simulink model "MMC_indc"  (R2026a)
settings: Solver=VariableStepAuto  StopTime=10
model workspace (MAT data in the model file):
  L_arm = 40
  L_arm_pow_rat = 14.4
  L_arm_res = 0.4
  L_arm_satcurrent = 7
  L_tolr = 15
  N = 8
  Rarm = 1
  Vdc = 375.5
libraries: nesl_utility x155, fl_lib x111, ee_lib x107
(part 1 of 14)
settings Model: Creator=tanus  LastModifiedBy=Shefali Pawgi
settings SimscapeCC: SimscapeNominalValues="[{\"value\":\"1\",\"unit\":\"A\"},{\"value\":\"1\",\"unit\":\"bar\"},{\"value\":\"1\",\"unit\":\"cm^2\"},{\"value\":\"1\",\"unit\":\"cm^3/s\"},{\"value\":\"1\",\"unit\":\"kJ/kg\"},{\"value\":\"1\",\"unit\":\"kW\"},{\"value\":\"1\",\"unit\":\"l\"},{\"value\":\"1\",\"unit\":\"N\"},{\"value\":\"1\",\"unit\":\"N*m\"},{\"value\":\"1\",\"unit\":\"V\"}]"  SimscapeLogType=none  SimscapeLogDataHistory=5000.0

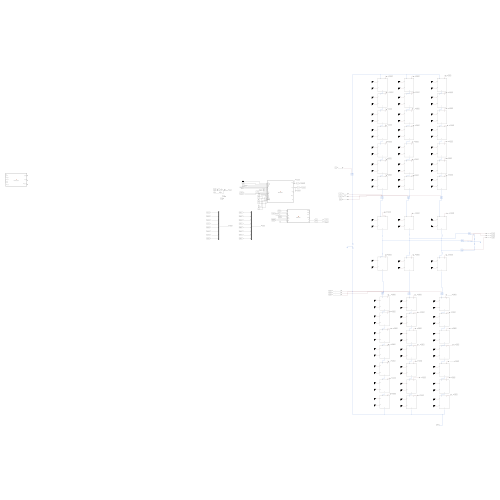
[thumbnail: Simulink's stored preview of the top-level diagram]
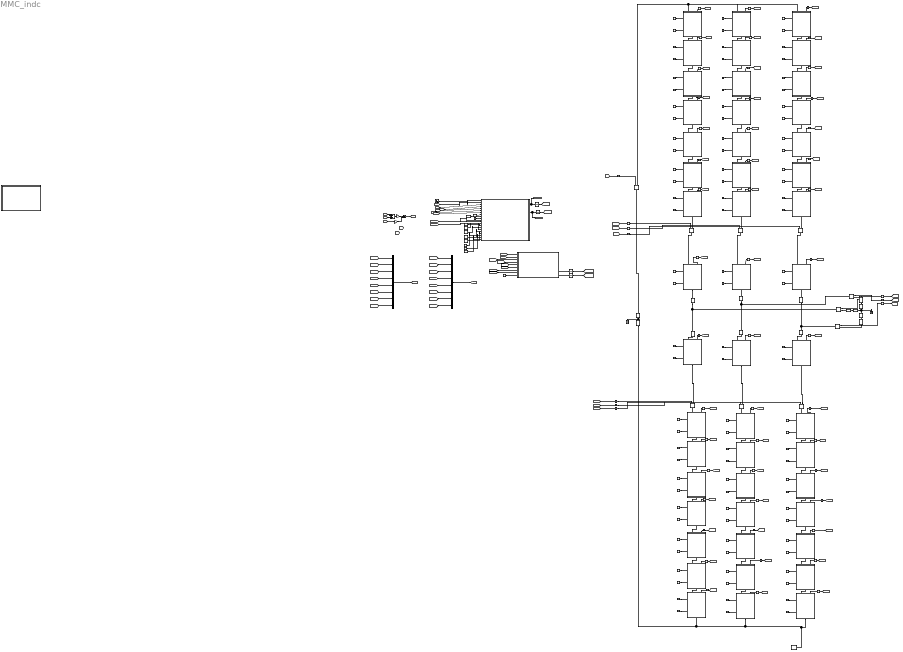
== system MMC_indc ==
  Constant : Constant  Value=Vdc
  Constant1 : Constant  Value=N
  Constant10 : Constant  Value=0.3
  Constant11 : Constant  Value=8
  Constant2 : Constant  Value=20e-3
  Constant3 : Constant  Value=10
  Constant4 : Constant  Value=220e-6
  Constant5 : Constant  Value=0.04
  Constant6 : Constant  Value=100e-3
  Constant7 : Constant
  Constant8 : Constant  Value=0.1
  Constant9 : Constant  Value=0.1
  Current Sensor{,1..9} (10 alike) : fl_lib/Electrical/Electrical Sensors/Current Sensor
  Electrical Reference : fl_lib/Electrical/Electrical Elements/Electrical Reference
  Electrical Reference1 : fl_lib/Electrical/Electrical Elements/Electrical Reference
  Gain : Gain  Gain=0.5
  Gain1 : Gain  Gain=1/3
  Inductor{1..4,6..7} (6 alike) : ee_lib/Passive/Inductor  l=L_arm mH  enable_L_tol=ee.enum.toleranceApplication.applyRand  L_tol=L_tolr  tol_distribution=ee.enum.toleranceDistribution.uniform  nSigma=4  r=L_arm_res Ohm  g=1e-9 1/Ohm  enable_operating_limits=ee.enum.enable.yes  operating_limit_action=ee.enum.passive.reportOpLim.warn  max_working_current=L_arm_satcurrent A  power_rating=L_arm_pow_rat W  i_L_specify=on  i_L_priority=High  i_L=0.44 A  i_L_nominal_specify=off  i_L_nominal_value=1  i_L_nominal_unit=A
  Inductor5 : ee_lib/Passive/Inductor  l=20e-3 H  enable_L_tol=ee.enum.toleranceApplication.none  L_tol=20  tol_distribution=ee.enum.toleranceDistribution.uniform  nSigma=4  r=0 Ohm  g=1e-9 1/Ohm  enable_operating_limits=ee.enum.enable.no  operating_limit_action=ee.enum.passive.reportOpLim.warn  max_working_current=1 A  power_rating=1 W  i_L_specify=on  i_L_priority=High  i_L=0.44 A  i_L_nominal_specify=off  i_L_nominal_value=1  i_L_nominal_unit=A
  Inductor8 : ee_lib/Passive/Inductor  l=20e-3 H  enable_L_tol=ee.enum.toleranceApplication.none  L_tol=20  tol_distribution=ee.enum.toleranceDistribution.uniform  nSigma=4  r=0 Ohm  g=1e-9 1/Ohm  enable_operating_limits=ee.enum.enable.no  operating_limit_action=ee.enum.passive.reportOpLim.warn  max_working_current=1 A  power_rating=1 W  i_L_specify=on  i_L_priority=High  i_L=0.44 A  i_L_nominal_specify=off  i_L_nominal_value=1  i_L_nominal_unit=A
  Inductor9 : ee_lib/Passive/Inductor  l=20e-3 H  enable_L_tol=ee.enum.toleranceApplication.none  L_tol=20  tol_distribution=ee.enum.toleranceDistribution.uniform  nSigma=4  r=0 Ohm  g=1e-9 1/Ohm  enable_operating_limits=ee.enum.enable.no  operating_limit_action=ee.enum.passive.reportOpLim.warn  max_working_current=1 A  power_rating=1 W  i_L_specify=on  i_L_priority=High  i_L=0.44 A  i_L_nominal_specify=off  i_L_nominal_value=1  i_L_nominal_unit=A
  MATLAB Function : MATLAB Function  TreatAsAtomicUnit=on
  MATLAB Function1 : MATLAB Function  TreatAsAtomicUnit=on
  MATLAB Function2 : MATLAB Function  TreatAsAtomicUnit=on
  Mux : Mux  Inputs=8
  Mux1 : Mux  Inputs=8
  PS-Simulink Converter{,1..57} (58 alike) : nesl_utility/PS-Simulink Converter  PhysicalDomain=network_engine_domain  SubClassName=ps_output  LeftPortType=input  RightPortType=output  PseudoPeriodic=off  Frequencies=[]  VectorFormat=inherit  Unit=inherit  AffineConversion=off
  Rarm : Constant  Value=0.4
  Resistor : fl_lib/Electrical/Electrical Elements/Resistor  R=10 Ohm  i_specify=off  i_priority=None  i=0 A  i_nominal_specify=off  i_nominal_value=1  i_nominal_unit=A  v_specify=off  v_priority=None  v=0 V  v_nominal_specify=off  v_nominal_value=1  v_nominal_unit=V
  Resistor1 : fl_lib/Electrical/Electrical Elements/Resistor  R=10 Ohm  i_specify=off  i_priority=None  i=0 A  i_nominal_specify=off  i_nominal_value=1  i_nominal_unit=A  v_specify=off  v_priority=None  v=0 V  v_nominal_specify=off  v_nominal_value=1  v_nominal_unit=V
  Resistor2 : fl_lib/Electrical/Electrical Elements/Resistor  R=10 Ohm  i_specify=off  i_priority=None  i=0 A  i_nominal_specify=off  i_nominal_value=1  i_nominal_unit=A  v_specify=off  v_priority=None  v=0 V  v_nominal_specify=off  v_nominal_value=1  v_nominal_unit=V
  Simulink-PS Converter{3..4,7..8,10..25,27..28,30..38,40..64,66..71,73..77,79..82,84..108} (96 alike) : nesl_utility/Simulink-PS Converter  PhysicalDomain=network_engine_domain  SubClassName=ps_input  LeftPortType=input  RightPortType=output  PseudoPeriodic=off  Frequencies=[]  NoiseDistribution=none  NoiseParameters=[]  Unit=1  AffineConversion=off  FilteringAndDerivatives=provide  SimscapeFilterOrder=1  InputFilterTimeConstant=0.001  UdotUserProvided=0
  Solver Configuration1 : nesl_utility/Solver Configuration  PhysicalDomain=network_engine_domain  SubClassName=solver  LeftPortType=input  RightPortType=generic  Tones=[]  Harmonics=[]  SimulateNoise=off  Profile=off  UseLocalSampling=off  EnableSwitchedLinearOptims=on  FrequencyDomain=off  UseCCode=off  RelTol=0.001  AbsTol=0.001  MinStep=1e-09  ToWorkspace=off  RevertToSquareIcSolve=off  NumHomotopyIterations=100  PhasorMode=off  PhasorModeNumHarmonics=1  ConsistencySolver=NEWTON_XTOL_AFTER_FTOL  CanonicalOrdering=UNORDERED  OptimizeIntermediates=UNOPTIMIZED  IndexReductionMethod=DerivativeReplacement  DoDC=off  ResidualTolerance=1e-09  ConsistencyTolSource=GLOBAL  ConsistencyAbsTol=0.001  ConsistencyRelTol=0.001  ConsistencyTolFactor=0.001  UseLocalSolver=off  LocalSolverChoice=NE_BACKWARD_EULER_ADVANCER  ResolveIndetEquations=on  FunctionEvalNumThread=1  LocalSolverSampleTime=0.001  DoFixedCost=off  MaxNonlinIter=3  MaxModeIter=2  ComputeImpulses=off  ImpulseIterations=2  LinearAlgebra=auto  LinearAlgebraNumThread=0  EquationFormulation=NE_TIME_EF  DelaysMemoryBudget=1024  AutomaticFiltering=on  FilteringTimeConstant=0.001  PartitionStorageMethod=AS_NEEDED  PartitionMemoryBudget=1024  PartitionMethod=ROBUST  MultibodyUseLocalSolver=off  MultibodyLocalSolverChoice=ODE1  MultibodyLocalSolverSampleTime=0.001
  Subsystem1 : Subsystem
      settings: PortSchema="{\"entries\":[{\"content\":{\"sides\":[{\"content\":{\"connectorIds\":[\"LConn1\",\"LConn2\"]},\"type\":\"ConnectorPlacement.EquallySpacedRectSide\",\"uuid\":\"15b6a701-c482-4ab4-b894-e969b74b8fe7\"},{\"content\":{\"side\":\"RIGHT\"},\"type\":\"ConnectorPlacement.EquallySpacedRectSide\",\"uuid\":\"d0e695dd-06b6-4831-9b12-69abc92aa4b4\"},{\"content\":{\"connectorIds\":[\"LConn3\",\"LConn4\"],\"side\":\"TOP\"},\"type\":\"ConnectorPlacement.EquallySpacedRectSide\",\"uuid\":\"2d8cca64-5216-4108-8582-3d735b4d6af0\"},{\"content\":{\"connectorIds\":[\"RConn1\"],\"side\":\"BOTTOM\"},\"type\":\"ConnectorPlacement.EquallySpacedRectSide\",\"uuid\":\"da22ed5b-3a7b-44e1-acef-3ebda742cad5\"}]},\"type\":\"ConnectorPlacement.EquallySpacedConnector\",\"uuid\":\"49f96526-0040-486f-9e93-d2a8b3aa1224\"}],\"packageUris\":[\"http://schema.mathworks.com/mf0/Connector/R2020b\"],\"version\":\"1.0\"}"
  Subsystem10 : Subsystem
      settings: PortSchema="{\"entries\":[{\"content\":{\"sides\":[{\"content\":{\"connectorIds\":[\"LConn1\",\"LConn2\"]},\"type\":\"ConnectorPlacement.EquallySpacedRectSide\",\"uuid\":\"15b6a701-c482-4ab4-b894-e969b74b8fe7\"},{\"content\":{\"side\":\"RIGHT\"},\"type\":\"ConnectorPlacement.EquallySpacedRectSide\",\"uuid\":\"d0e695dd-06b6-4831-9b12-69abc92aa4b4\"},{\"content\":{\"connectorIds\":[\"LConn3\",\"LConn4\"],\"side\":\"TOP\"},\"type\":\"ConnectorPlacement.EquallySpacedRectSide\",\"uuid\":\"2d8cca64-5216-4108-8582-3d735b4d6af0\"},{\"content\":{\"connectorIds\":[\"RConn1\"],\"side\":\"BOTTOM\"},\"type\":\"ConnectorPlacement.EquallySpacedRectSide\",\"uuid\":\"da22ed5b-3a7b-44e1-acef-3ebda742cad5\"}]},\"type\":\"ConnectorPlacement.EquallySpacedConnector\",\"uuid\":\"49f96526-0040-486f-9e93-d2a8b3aa1224\"}],\"packageUris\":[\"http://schema.mathworks.com/mf0/Connector/R2020b\"],\"version\":\"1.0\"}"
  Subsystem11 : Subsystem
      settings: PortSchema="{\"entries\":[{\"content\":{\"sides\":[{\"content\":{\"connectorIds\":[\"LConn1\",\"LConn2\"]},\"type\":\"ConnectorPlacement.EquallySpacedRectSide\",\"uuid\":\"15b6a701-c482-4ab4-b894-e969b74b8fe7\"},{\"content\":{\"side\":\"RIGHT\"},\"type\":\"ConnectorPlacement.EquallySpacedRectSide\",\"uuid\":\"d0e695dd-06b6-4831-9b12-69abc92aa4b4\"},{\"content\":{\"connectorIds\":[\"LConn3\",\"LConn4\"],\"side\":\"TOP\"},\"type\":\"ConnectorPlacement.EquallySpacedRectSide\",\"uuid\":\"2d8cca64-5216-4108-8582-3d735b4d6af0\"},{\"content\":{\"connectorIds\":[\"RConn1\"],\"side\":\"BOTTOM\"},\"type\":\"ConnectorPlacement.EquallySpacedRectSide\",\"uuid\":\"da22ed5b-3a7b-44e1-acef-3ebda742cad5\"}]},\"type\":\"ConnectorPlacement.EquallySpacedConnector\",\"uuid\":\"49f96526-0040-486f-9e93-d2a8b3aa1224\"}],\"packageUris\":[\"http://schema.mathworks.com/mf0/Connector/R2020b\"],\"version\":\"1.0\"}"
  Subsystem12 : Subsystem
      settings: PortSchema="{\"entries\":[{\"content\":{\"sides\":[{\"content\":{\"connectorIds\":[\"LConn1\",\"LConn2\"]},\"type\":\"ConnectorPlacement.EquallySpacedRectSide\",\"uuid\":\"15b6a701-c482-4ab4-b894-e969b74b8fe7\"},{\"content\":{\"side\":\"RIGHT\"},\"type\":\"ConnectorPlacement.EquallySpacedRectSide\",\"uuid\":\"d0e695dd-06b6-4831-9b12-69abc92aa4b4\"},{\"content\":{\"connectorIds\":[\"LConn3\",\"LConn4\"],\"side\":\"TOP\"},\"type\":\"ConnectorPlacement.EquallySpacedRectSide\",\"uuid\":\"2d8cca64-5216-4108-8582-3d735b4d6af0\"},{\"content\":{\"connectorIds\":[\"RConn1\"],\"side\":\"BOTTOM\"},\"type\":\"ConnectorPlacement.EquallySpacedRectSide\",\"uuid\":\"da22ed5b-3a7b-44e1-acef-3ebda742cad5\"}]},\"type\":\"ConnectorPlacement.EquallySpacedConnector\",\"uuid\":\"49f96526-0040-486f-9e93-d2a8b3aa1224\"}],\"packageUris\":[\"http://schema.mathworks.com/mf0/Connector/R2020b\"],\"version\":\"1.0\"}"
  Subsystem13 : Subsystem
      settings: PortSchema="{\"entries\":[{\"content\":{\"sides\":[{\"content\":{\"connectorIds\":[\"LConn1\",\"LConn2\"]},\"type\":\"ConnectorPlacement.EquallySpacedRectSide\",\"uuid\":\"15b6a701-c482-4ab4-b894-e969b74b8fe7\"},{\"content\":{\"side\":\"RIGHT\"},\"type\":\"ConnectorPlacement.EquallySpacedRectSide\",\"uuid\":\"d0e695dd-06b6-4831-9b12-69abc92aa4b4\"},{\"content\":{\"connectorIds\":[\"LConn3\",\"LConn4\"],\"side\":\"TOP\"},\"type\":\"ConnectorPlacement.EquallySpacedRectSide\",\"uuid\":\"2d8cca64-5216-4108-8582-3d735b4d6af0\"},{\"content\":{\"connectorIds\":[\"RConn1\"],\"side\":\"BOTTOM\"},\"type\":\"ConnectorPlacement.EquallySpacedRectSide\",\"uuid\":\"da22ed5b-3a7b-44e1-acef-3ebda742cad5\"}]},\"type\":\"ConnectorPlacement.EquallySpacedConnector\",\"uuid\":\"49f96526-0040-486f-9e93-d2a8b3aa1224\"}],\"packageUris\":[\"http://schema.mathworks.com/mf0/Connector/R2020b\"],\"version\":\"1.0\"}"
  Subsystem14 : Subsystem
      settings: PortSchema="{\"entries\":[{\"content\":{\"sides\":[{\"content\":{\"connectorIds\":[\"LConn1\",\"LConn2\"]},\"type\":\"ConnectorPlacement.EquallySpacedRectSide\",\"uuid\":\"15b6a701-c482-4ab4-b894-e969b74b8fe7\"},{\"content\":{\"side\":\"RIGHT\"},\"type\":\"ConnectorPlacement.EquallySpacedRectSide\",\"uuid\":\"d0e695dd-06b6-4831-9b12-69abc92aa4b4\"},{\"content\":{\"connectorIds\":[\"LConn3\",\"LConn4\"],\"side\":\"TOP\"},\"type\":\"ConnectorPlacement.EquallySpacedRectSide\",\"uuid\":\"2d8cca64-5216-4108-8582-3d735b4d6af0\"},{\"content\":{\"connectorIds\":[\"RConn1\"],\"side\":\"BOTTOM\"},\"type\":\"ConnectorPlacement.EquallySpacedRectSide\",\"uuid\":\"da22ed5b-3a7b-44e1-acef-3ebda742cad5\"}]},\"type\":\"ConnectorPlacement.EquallySpacedConnector\",\"uuid\":\"49f96526-0040-486f-9e93-d2a8b3aa1224\"}],\"packageUris\":[\"http://schema.mathworks.com/mf0/Connector/R2020b\"],\"version\":\"1.0\"}"
  Subsystem16 : Subsystem
      settings: PortSchema="{\"entries\":[{\"content\":{\"sides\":[{\"content\":{\"connectorIds\":[\"LConn1\",\"LConn2\"]},\"type\":\"ConnectorPlacement.EquallySpacedRectSide\",\"uuid\":\"15b6a701-c482-4ab4-b894-e969b74b8fe7\"},{\"content\":{\"side\":\"RIGHT\"},\"type\":\"ConnectorPlacement.EquallySpacedRectSide\",\"uuid\":\"d0e695dd-06b6-4831-9b12-69abc92aa4b4\"},{\"content\":{\"connectorIds\":[\"LConn3\",\"LConn4\"],\"side\":\"TOP\"},\"type\":\"ConnectorPlacement.EquallySpacedRectSide\",\"uuid\":\"2d8cca64-5216-4108-8582-3d735b4d6af0\"},{\"content\":{\"connectorIds\":[\"RConn1\"],\"side\":\"BOTTOM\"},\"type\":\"ConnectorPlacement.EquallySpacedRectSide\",\"uuid\":\"da22ed5b-3a7b-44e1-acef-3ebda742cad5\"}]},\"type\":\"ConnectorPlacement.EquallySpacedConnector\",\"uuid\":\"49f96526-0040-486f-9e93-d2a8b3aa1224\"}],\"packageUris\":[\"http://schema.mathworks.com/mf0/Connector/R2020b\"],\"version\":\"1.0\"}"
  Subsystem17 : Subsystem
      settings: PortSchema="{\"entries\":[{\"content\":{\"sides\":[{\"content\":{\"connectorIds\":[\"LConn1\",\"LConn2\"]},\"type\":\"ConnectorPlacement.EquallySpacedRectSide\",\"uuid\":\"15b6a701-c482-4ab4-b894-e969b74b8fe7\"},{\"content\":{\"side\":\"RIGHT\"},\"type\":\"ConnectorPlacement.EquallySpacedRectSide\",\"uuid\":\"d0e695dd-06b6-4831-9b12-69abc92aa4b4\"},{\"content\":{\"connectorIds\":[\"LConn3\",\"LConn4\"],\"side\":\"TOP\"},\"type\":\"ConnectorPlacement.EquallySpacedRectSide\",\"uuid\":\"2d8cca64-5216-4108-8582-3d735b4d6af0\"},{\"content\":{\"connectorIds\":[\"RConn1\"],\"side\":\"BOTTOM\"},\"type\":\"ConnectorPlacement.EquallySpacedRectSide\",\"uuid\":\"da22ed5b-3a7b-44e1-acef-3ebda742cad5\"}]},\"type\":\"ConnectorPlacement.EquallySpacedConnector\",\"uuid\":\"49f96526-0040-486f-9e93-d2a8b3aa1224\"}],\"packageUris\":[\"http://schema.mathworks.com/mf0/Connector/R2020b\"],\"version\":\"1.0\"}"
  Subsystem18 : Subsystem
      settings: PortSchema="{\"entries\":[{\"content\":{\"sides\":[{\"content\":{\"connectorIds\":[\"LConn1\",\"LConn2\"]},\"type\":\"ConnectorPlacement.EquallySpacedRectSide\",\"uuid\":\"15b6a701-c482-4ab4-b894-e969b74b8fe7\"},{\"content\":{\"side\":\"RIGHT\"},\"type\":\"ConnectorPlacement.EquallySpacedRectSide\",\"uuid\":\"d0e695dd-06b6-4831-9b12-69abc92aa4b4\"},{\"content\":{\"connectorIds\":[\"LConn3\",\"LConn4\"],\"side\":\"TOP\"},\"type\":\"ConnectorPlacement.EquallySpacedRectSide\",\"uuid\":\"2d8cca64-5216-4108-8582-3d735b4d6af0\"},{\"content\":{\"connectorIds\":[\"RConn1\"],\"side\":\"BOTTOM\"},\"type\":\"ConnectorPlacement.EquallySpacedRectSide\",\"uuid\":\"da22ed5b-3a7b-44e1-acef-3ebda742cad5\"}]},\"type\":\"ConnectorPlacement.EquallySpacedConnector\",\"uuid\":\"49f96526-0040-486f-9e93-d2a8b3aa1224\"}],\"packageUris\":[\"http://schema.mathworks.com/mf0/Connector/R2020b\"],\"version\":\"1.0\"}"
  Subsystem19 : Subsystem
      settings: PortSchema="{\"entries\":[{\"content\":{\"sides\":[{\"content\":{\"connectorIds\":[\"LConn1\",\"LConn2\"]},\"type\":\"ConnectorPlacement.EquallySpacedRectSide\",\"uuid\":\"15b6a701-c482-4ab4-b894-e969b74b8fe7\"},{\"content\":{\"side\":\"RIGHT\"},\"type\":\"ConnectorPlacement.EquallySpacedRectSide\",\"uuid\":\"d0e695dd-06b6-4831-9b12-69abc92aa4b4\"},{\"content\":{\"connectorIds\":[\"LConn3\",\"LConn4\"],\"side\":\"TOP\"},\"type\":\"ConnectorPlacement.EquallySpacedRectSide\",\"uuid\":\"2d8cca64-5216-4108-8582-3d735b4d6af0\"},{\"content\":{\"connectorIds\":[\"RConn1\"],\"side\":\"BOTTOM\"},\"type\":\"ConnectorPlacement.EquallySpacedRectSide\",\"uuid\":\"da22ed5b-3a7b-44e1-acef-3ebda742cad5\"}]},\"type\":\"ConnectorPlacement.EquallySpacedConnector\",\"uuid\":\"49f96526-0040-486f-9e93-d2a8b3aa1224\"}],\"packageUris\":[\"http://schema.mathworks.com/mf0/Connector/R2020b\"],\"version\":\"1.0\"}"
  Subsystem2 : Subsystem
      settings: PortSchema="{\"entries\":[{\"content\":{\"sides\":[{\"content\":{\"connectorIds\":[\"LConn1\",\"LConn2\"]},\"type\":\"ConnectorPlacement.EquallySpacedRectSide\",\"uuid\":\"15b6a701-c482-4ab4-b894-e969b74b8fe7\"},{\"content\":{\"side\":\"RIGHT\"},\"type\":\"ConnectorPlacement.EquallySpacedRectSide\",\"uuid\":\"d0e695dd-06b6-4831-9b12-69abc92aa4b4\"},{\"content\":{\"connectorIds\":[\"LConn3\",\"LConn4\"],\"side\":\"TOP\"},\"type\":\"ConnectorPlacement.EquallySpacedRectSide\",\"uuid\":\"2d8cca64-5216-4108-8582-3d735b4d6af0\"},{\"content\":{\"connectorIds\":[\"RConn1\"],\"side\":\"BOTTOM\"},\"type\":\"ConnectorPlacement.EquallySpacedRectSide\",\"uuid\":\"da22ed5b-3a7b-44e1-acef-3ebda742cad5\"}]},\"type\":\"ConnectorPlacement.EquallySpacedConnector\",\"uuid\":\"49f96526-0040-486f-9e93-d2a8b3aa1224\"}],\"packageUris\":[\"http://schema.mathworks.com/mf0/Connector/R2020b\"],\"version\":\"1.0\"}"
  Subsystem20 : Subsystem
      settings: PortSchema="{\"entries\":[{\"content\":{\"sides\":[{\"content\":{\"connectorIds\":[\"LConn1\",\"LConn2\"]},\"type\":\"ConnectorPlacement.EquallySpacedRectSide\",\"uuid\":\"15b6a701-c482-4ab4-b894-e969b74b8fe7\"},{\"content\":{\"side\":\"RIGHT\"},\"type\":\"ConnectorPlacement.EquallySpacedRectSide\",\"uuid\":\"d0e695dd-06b6-4831-9b12-69abc92aa4b4\"},{\"content\":{\"connectorIds\":[\"LConn3\",\"LConn4\"],\"side\":\"TOP\"},\"type\":\"ConnectorPlacement.EquallySpacedRectSide\",\"uuid\":\"2d8cca64-5216-4108-8582-3d735b4d6af0\"},{\"content\":{\"connectorIds\":[\"RConn1\"],\"side\":\"BOTTOM\"},\"type\":\"ConnectorPlacement.EquallySpacedRectSide\",\"uuid\":\"da22ed5b-3a7b-44e1-acef-3ebda742cad5\"}]},\"type\":\"ConnectorPlacement.EquallySpacedConnector\",\"uuid\":\"49f96526-0040-486f-9e93-d2a8b3aa1224\"}],\"packageUris\":[\"http://schema.mathworks.com/mf0/Connector/R2020b\"],\"version\":\"1.0\"}"
  Subsystem21 : Subsystem
      settings: PortSchema="{\"entries\":[{\"content\":{\"sides\":[{\"content\":{\"connectorIds\":[\"LConn1\",\"LConn2\"]},\"type\":\"ConnectorPlacement.EquallySpacedRectSide\",\"uuid\":\"15b6a701-c482-4ab4-b894-e969b74b8fe7\"},{\"content\":{\"side\":\"RIGHT\"},\"type\":\"ConnectorPlacement.EquallySpacedRectSide\",\"uuid\":\"d0e695dd-06b6-4831-9b12-69abc92aa4b4\"},{\"content\":{\"connectorIds\":[\"LConn3\",\"LConn4\"],\"side\":\"TOP\"},\"type\":\"ConnectorPlacement.EquallySpacedRectSide\",\"uuid\":\"2d8cca64-5216-4108-8582-3d735b4d6af0\"},{\"content\":{\"connectorIds\":[\"RConn1\"],\"side\":\"BOTTOM\"},\"type\":\"ConnectorPlacement.EquallySpacedRectSide\",\"uuid\":\"da22ed5b-3a7b-44e1-acef-3ebda742cad5\"}]},\"type\":\"ConnectorPlacement.EquallySpacedConnector\",\"uuid\":\"49f96526-0040-486f-9e93-d2a8b3aa1224\"}],\"packageUris\":[\"http://schema.mathworks.com/mf0/Connector/R2020b\"],\"version\":\"1.0\"}"
  Subsystem22 : Subsystem
      settings: PortSchema="{\"entries\":[{\"content\":{\"sides\":[{\"content\":{\"connectorIds\":[\"LConn1\",\"LConn2\"]},\"type\":\"ConnectorPlacement.EquallySpacedRectSide\",\"uuid\":\"15b6a701-c482-4ab4-b894-e969b74b8fe7\"},{\"content\":{\"side\":\"RIGHT\"},\"type\":\"ConnectorPlacement.EquallySpacedRectSide\",\"uuid\":\"d0e695dd-06b6-4831-9b12-69abc92aa4b4\"},{\"content\":{\"connectorIds\":[\"LConn3\",\"LConn4\"],\"side\":\"TOP\"},\"type\":\"ConnectorPlacement.EquallySpacedRectSide\",\"uuid\":\"2d8cca64-5216-4108-8582-3d735b4d6af0\"},{\"content\":{\"connectorIds\":[\"RConn1\"],\"side\":\"BOTTOM\"},\"type\":\"ConnectorPlacement.EquallySpacedRectSide\",\"uuid\":\"da22ed5b-3a7b-44e1-acef-3ebda742cad5\"}]},\"type\":\"ConnectorPlacement.EquallySpacedConnector\",\"uuid\":\"49f96526-0040-486f-9e93-d2a8b3aa1224\"}],\"packageUris\":[\"http://schema.mathworks.com/mf0/Connector/R2020b\"],\"version\":\"1.0\"}"
  Subsystem23 : Subsystem
      settings: PortSchema="{\"entries\":[{\"content\":{\"sides\":[{\"content\":{\"connectorIds\":[\"LConn1\",\"LConn2\"]},\"type\":\"ConnectorPlacement.EquallySpacedRectSide\",\"uuid\":\"15b6a701-c482-4ab4-b894-e969b74b8fe7\"},{\"content\":{\"side\":\"RIGHT\"},\"type\":\"ConnectorPlacement.EquallySpacedRectSide\",\"uuid\":\"d0e695dd-06b6-4831-9b12-69abc92aa4b4\"},{\"content\":{\"connectorIds\":[\"LConn3\",\"LConn4\"],\"side\":\"TOP\"},\"type\":\"ConnectorPlacement.EquallySpacedRectSide\",\"uuid\":\"2d8cca64-5216-4108-8582-3d735b4d6af0\"},{\"content\":{\"connectorIds\":[\"RConn1\"],\"side\":\"BOTTOM\"},\"type\":\"ConnectorPlacement.EquallySpacedRectSide\",\"uuid\":\"da22ed5b-3a7b-44e1-acef-3ebda742cad5\"}]},\"type\":\"ConnectorPlacement.EquallySpacedConnector\",\"uuid\":\"49f96526-0040-486f-9e93-d2a8b3aa1224\"}],\"packageUris\":[\"http://schema.mathworks.com/mf0/Connector/R2020b\"],\"version\":\"1.0\"}"
  Subsystem24 : Subsystem
      settings: PortSchema="{\"entries\":[{\"content\":{\"sides\":[{\"content\":{\"connectorIds\":[\"LConn1\",\"LConn2\"]},\"type\":\"ConnectorPlacement.EquallySpacedRectSide\",\"uuid\":\"15b6a701-c482-4ab4-b894-e969b74b8fe7\"},{\"content\":{\"side\":\"RIGHT\"},\"type\":\"ConnectorPlacement.EquallySpacedRectSide\",\"uuid\":\"d0e695dd-06b6-4831-9b12-69abc92aa4b4\"},{\"content\":{\"connectorIds\":[\"LConn3\",\"LConn4\"],\"side\":\"TOP\"},\"type\":\"ConnectorPlacement.EquallySpacedRectSide\",\"uuid\":\"2d8cca64-5216-4108-8582-3d735b4d6af0\"},{\"content\":{\"connectorIds\":[\"RConn1\"],\"side\":\"BOTTOM\"},\"type\":\"ConnectorPlacement.EquallySpacedRectSide\",\"uuid\":\"da22ed5b-3a7b-44e1-acef-3ebda742cad5\"}]},\"type\":\"ConnectorPlacement.EquallySpacedConnector\",\"uuid\":\"49f96526-0040-486f-9e93-d2a8b3aa1224\"}],\"packageUris\":[\"http://schema.mathworks.com/mf0/Connector/R2020b\"],\"version\":\"1.0\"}"
  Subsystem25 : Subsystem
      settings: PortSchema="{\"entries\":[{\"content\":{\"sides\":[{\"content\":{\"connectorIds\":[\"LConn1\",\"LConn2\"]},\"type\":\"ConnectorPlacement.EquallySpacedRectSide\",\"uuid\":\"15b6a701-c482-4ab4-b894-e969b74b8fe7\"},{\"content\":{\"side\":\"RIGHT\"},\"type\":\"ConnectorPlacement.EquallySpacedRectSide\",\"uuid\":\"d0e695dd-06b6-4831-9b12-69abc92aa4b4\"},{\"content\":{\"connectorIds\":[\"LConn3\",\"LConn4\"],\"side\":\"TOP\"},\"type\":\"ConnectorPlacement.EquallySpacedRectSide\",\"uuid\":\"2d8cca64-5216-4108-8582-3d735b4d6af0\"},{\"content\":{\"connectorIds\":[\"RConn1\"],\"side\":\"BOTTOM\"},\"type\":\"ConnectorPlacement.EquallySpacedRectSide\",\"uuid\":\"da22ed5b-3a7b-44e1-acef-3ebda742cad5\"}]},\"type\":\"ConnectorPlacement.EquallySpacedConnector\",\"uuid\":\"49f96526-0040-486f-9e93-d2a8b3aa1224\"}],\"packageUris\":[\"http://schema.mathworks.com/mf0/Connector/R2020b\"],\"version\":\"1.0\"}"
  Subsystem26 : Subsystem
      settings: PortSchema="{\"entries\":[{\"content\":{\"sides\":[{\"content\":{\"connectorIds\":[\"LConn1\",\"LConn2\"]},\"type\":\"ConnectorPlacement.EquallySpacedRectSide\",\"uuid\":\"15b6a701-c482-4ab4-b894-e969b74b8fe7\"},{\"content\":{\"side\":\"RIGHT\"},\"type\":\"ConnectorPlacement.EquallySpacedRectSide\",\"uuid\":\"d0e695dd-06b6-4831-9b12-69abc92aa4b4\"},{\"content\":{\"connectorIds\":[\"LConn3\",\"LConn4\"],\"side\":\"TOP\"},\"type\":\"ConnectorPlacement.EquallySpacedRectSide\",\"uuid\":\"2d8cca64-5216-4108-8582-3d735b4d6af0\"},{\"content\":{\"connectorIds\":[\"RConn1\"],\"side\":\"BOTTOM\"},\"type\":\"ConnectorPlacement.EquallySpacedRectSide\",\"uuid\":\"da22ed5b-3a7b-44e1-acef-3ebda742cad5\"}]},\"type\":\"ConnectorPlacement.EquallySpacedConnector\",\"uuid\":\"49f96526-0040-486f-9e93-d2a8b3aa1224\"}],\"packageUris\":[\"http://schema.mathworks.com/mf0/Connector/R2020b\"],\"version\":\"1.0\"}"
  Subsystem27 : Subsystem
      settings: PortSchema="{\"entries\":[{\"content\":{\"sides\":[{\"content\":{\"connectorIds\":[\"LConn1\",\"LConn2\"]},\"type\":\"ConnectorPlacement.EquallySpacedRectSide\",\"uuid\":\"15b6a701-c482-4ab4-b894-e969b74b8fe7\"},{\"content\":{\"side\":\"RIGHT\"},\"type\":\"ConnectorPlacement.EquallySpacedRectSide\",\"uuid\":\"d0e695dd-06b6-4831-9b12-69abc92aa4b4\"},{\"content\":{\"connectorIds\":[\"LConn3\",\"LConn4\"],\"side\":\"TOP\"},\"type\":\"ConnectorPlacement.EquallySpacedRectSide\",\"uuid\":\"2d8cca64-5216-4108-8582-3d735b4d6af0\"},{\"content\":{\"connectorIds\":[\"RConn1\"],\"side\":\"BOTTOM\"},\"type\":\"ConnectorPlacement.EquallySpacedRectSide\",\"uuid\":\"da22ed5b-3a7b-44e1-acef-3ebda742cad5\"}]},\"type\":\"ConnectorPlacement.EquallySpacedConnector\",\"uuid\":\"49f96526-0040-486f-9e93-d2a8b3aa1224\"}],\"packageUris\":[\"http://schema.mathworks.com/mf0/Connector/R2020b\"],\"version\":\"1.0\"}"
  Subsystem28 : Subsystem
      settings: PortSchema="{\"entries\":[{\"content\":{\"sides\":[{\"content\":{\"connectorIds\":[\"LConn1\",\"LConn2\"]},\"type\":\"ConnectorPlacement.EquallySpacedRectSide\",\"uuid\":\"15b6a701-c482-4ab4-b894-e969b74b8fe7\"},{\"content\":{\"side\":\"RIGHT\"},\"type\":\"ConnectorPlacement.EquallySpacedRectSide\",\"uuid\":\"d0e695dd-06b6-4831-9b12-69abc92aa4b4\"},{\"content\":{\"connectorIds\":[\"LConn3\",\"LConn4\"],\"side\":\"TOP\"},\"type\":\"ConnectorPlacement.EquallySpacedRectSide\",\"uuid\":\"2d8cca64-5216-4108-8582-3d735b4d6af0\"},{\"content\":{\"connectorIds\":[\"RConn1\"],\"side\":\"BOTTOM\"},\"type\":\"ConnectorPlacement.EquallySpacedRectSide\",\"uuid\":\"da22ed5b-3a7b-44e1-acef-3ebda742cad5\"}]},\"type\":\"ConnectorPlacement.EquallySpacedConnector\",\"uuid\":\"49f96526-0040-486f-9e93-d2a8b3aa1224\"}],\"packageUris\":[\"http://schema.mathworks.com/mf0/Connector/R2020b\"],\"version\":\"1.0\"}"
  Subsystem3 : Subsystem
      settings: PortSchema="{\"entries\":[{\"content\":{\"sides\":[{\"content\":{\"connectorIds\":[\"LConn1\",\"LConn2\"]},\"type\":\"ConnectorPlacement.EquallySpacedRectSide\",\"uuid\":\"15b6a701-c482-4ab4-b894-e969b74b8fe7\"},{\"content\":{\"side\":\"RIGHT\"},\"type\":\"ConnectorPlacement.EquallySpacedRectSide\",\"uuid\":\"d0e695dd-06b6-4831-9b12-69abc92aa4b4\"},{\"content\":{\"connectorIds\":[\"LConn3\",\"LConn4\"],\"side\":\"TOP\"},\"type\":\"ConnectorPlacement.EquallySpacedRectSide\",\"uuid\":\"2d8cca64-5216-4108-8582-3d735b4d6af0\"},{\"content\":{\"connectorIds\":[\"RConn1\"],\"side\":\"BOTTOM\"},\"type\":\"ConnectorPlacement.EquallySpacedRectSide\",\"uuid\":\"da22ed5b-3a7b-44e1-acef-3ebda742cad5\"}]},\"type\":\"ConnectorPlacement.EquallySpacedConnector\",\"uuid\":\"49f96526-0040-486f-9e93-d2a8b3aa1224\"}],\"packageUris\":[\"http://schema.mathworks.com/mf0/Connector/R2020b\"],\"version\":\"1.0\"}"
  Subsystem30 : Subsystem
      settings: PortSchema="{\"entries\":[{\"content\":{\"sides\":[{\"content\":{\"connectorIds\":[\"LConn1\",\"LConn2\"]},\"type\":\"ConnectorPlacement.EquallySpacedRectSide\",\"uuid\":\"15b6a701-c482-4ab4-b894-e969b74b8fe7\"},{\"content\":{\"side\":\"RIGHT\"},\"type\":\"ConnectorPlacement.EquallySpacedRectSide\",\"uuid\":\"d0e695dd-06b6-4831-9b12-69abc92aa4b4\"},{\"content\":{\"connectorIds\":[\"LConn3\",\"LConn4\"],\"side\":\"TOP\"},\"type\":\"ConnectorPlacement.EquallySpacedRectSide\",\"uuid\":\"2d8cca64-5216-4108-8582-3d735b4d6af0\"},{\"content\":{\"connectorIds\":[\"RConn1\"],\"side\":\"BOTTOM\"},\"type\":\"ConnectorPlacement.EquallySpacedRectSide\",\"uuid\":\"da22ed5b-3a7b-44e1-acef-3ebda742cad5\"}]},\"type\":\"ConnectorPlacement.EquallySpacedConnector\",\"uuid\":\"49f96526-0040-486f-9e93-d2a8b3aa1224\"}],\"packageUris\":[\"http://schema.mathworks.com/mf0/Connector/R2020b\"],\"version\":\"1.0\"}"
  Subsystem31 : Subsystem
      settings: PortSchema="{\"entries\":[{\"content\":{\"sides\":[{\"content\":{\"connectorIds\":[\"LConn1\",\"LConn2\"]},\"type\":\"ConnectorPlacement.EquallySpacedRectSide\",\"uuid\":\"15b6a701-c482-4ab4-b894-e969b74b8fe7\"},{\"content\":{\"side\":\"RIGHT\"},\"type\":\"ConnectorPlacement.EquallySpacedRectSide\",\"uuid\":\"d0e695dd-06b6-4831-9b12-69abc92aa4b4\"},{\"content\":{\"connectorIds\":[\"LConn3\",\"LConn4\"],\"side\":\"TOP\"},\"type\":\"ConnectorPlacement.EquallySpacedRectSide\",\"uuid\":\"2d8cca64-5216-4108-8582-3d735b4d6af0\"},{\"content\":{\"connectorIds\":[\"RConn1\"],\"side\":\"BOTTOM\"},\"type\":\"ConnectorPlacement.EquallySpacedRectSide\",\"uuid\":\"da22ed5b-3a7b-44e1-acef-3ebda742cad5\"}]},\"type\":\"ConnectorPlacement.EquallySpacedConnector\",\"uuid\":\"49f96526-0040-486f-9e93-d2a8b3aa1224\"}],\"packageUris\":[\"http://schema.mathworks.com/mf0/Connector/R2020b\"],\"version\":\"1.0\"}"
  Subsystem33 : Subsystem
      settings: PortSchema="{\"entries\":[{\"content\":{\"sides\":[{\"content\":{\"connectorIds\":[\"LConn1\",\"LConn2\"]},\"type\":\"ConnectorPlacement.EquallySpacedRectSide\",\"uuid\":\"15b6a701-c482-4ab4-b894-e969b74b8fe7\"},{\"content\":{\"side\":\"RIGHT\"},\"type\":\"ConnectorPlacement.EquallySpacedRectSide\",\"uuid\":\"d0e695dd-06b6-4831-9b12-69abc92aa4b4\"},{\"content\":{\"connectorIds\":[\"LConn3\",\"LConn4\"],\"side\":\"TOP\"},\"type\":\"ConnectorPlacement.EquallySpacedRectSide\",\"uuid\":\"2d8cca64-5216-4108-8582-3d735b4d6af0\"},{\"content\":{\"connectorIds\":[\"RConn1\"],\"side\":\"BOTTOM\"},\"type\":\"ConnectorPlacement.EquallySpacedRectSide\",\"uuid\":\"da22ed5b-3a7b-44e1-acef-3ebda742cad5\"}]},\"type\":\"ConnectorPlacement.EquallySpacedConnector\",\"uuid\":\"49f96526-0040-486f-9e93-d2a8b3aa1224\"}],\"packageUris\":[\"http://schema.mathworks.com/mf0/Connector/R2020b\"],\"version\":\"1.0\"}"
  Subsystem34 : Subsystem
      settings: PortSchema="{\"entries\":[{\"content\":{\"sides\":[{\"content\":{\"connectorIds\":[\"LConn1\",\"LConn2\"]},\"type\":\"ConnectorPlacement.EquallySpacedRectSide\",\"uuid\":\"15b6a701-c482-4ab4-b894-e969b74b8fe7\"},{\"content\":{\"side\":\"RIGHT\"},\"type\":\"ConnectorPlacement.EquallySpacedRectSide\",\"uuid\":\"d0e695dd-06b6-4831-9b12-69abc92aa4b4\"},{\"content\":{\"connectorIds\":[\"LConn3\",\"LConn4\"],\"side\":\"TOP\"},\"type\":\"ConnectorPlacement.EquallySpacedRectSide\",\"uuid\":\"2d8cca64-5216-4108-8582-3d735b4d6af0\"},{\"content\":{\"connectorIds\":[\"RConn1\"],\"side\":\"BOTTOM\"},\"type\":\"ConnectorPlacement.EquallySpacedRectSide\",\"uuid\":\"da22ed5b-3a7b-44e1-acef-3ebda742cad5\"}]},\"type\":\"ConnectorPlacement.EquallySpacedConnector\",\"uuid\":\"49f96526-0040-486f-9e93-d2a8b3aa1224\"}],\"packageUris\":[\"http://schema.mathworks.com/mf0/Connector/R2020b\"],\"version\":\"1.0\"}"
  Subsystem35 : Subsystem
      settings: PortSchema="{\"entries\":[{\"content\":{\"sides\":[{\"content\":{\"connectorIds\":[\"LConn1\",\"LConn2\"]},\"type\":\"ConnectorPlacement.EquallySpacedRectSide\",\"uuid\":\"15b6a701-c482-4ab4-b894-e969b74b8fe7\"},{\"content\":{\"side\":\"RIGHT\"},\"type\":\"ConnectorPlacement.EquallySpacedRectSide\",\"uuid\":\"d0e695dd-06b6-4831-9b12-69abc92aa4b4\"},{\"content\":{\"connectorIds\":[\"LConn3\",\"LConn4\"],\"side\":\"TOP\"},\"type\":\"ConnectorPlacement.EquallySpacedRectSide\",\"uuid\":\"2d8cca64-5216-4108-8582-3d735b4d6af0\"},{\"content\":{\"connectorIds\":[\"RConn1\"],\"side\":\"BOTTOM\"},\"type\":\"ConnectorPlacement.EquallySpacedRectSide\",\"uuid\":\"da22ed5b-3a7b-44e1-acef-3ebda742cad5\"}]},\"type\":\"ConnectorPlacement.EquallySpacedConnector\",\"uuid\":\"49f96526-0040-486f-9e93-d2a8b3aa1224\"}],\"packageUris\":[\"http://schema.mathworks.com/mf0/Connector/R2020b\"],\"version\":\"1.0\"}"
  Subsystem36 : Subsystem
      settings: PortSchema="{\"entries\":[{\"content\":{\"sides\":[{\"content\":{\"connectorIds\":[\"LConn1\",\"LConn2\"]},\"type\":\"ConnectorPlacement.EquallySpacedRectSide\",\"uuid\":\"15b6a701-c482-4ab4-b894-e969b74b8fe7\"},{\"content\":{\"side\":\"RIGHT\"},\"type\":\"ConnectorPlacement.EquallySpacedRectSide\",\"uuid\":\"d0e695dd-06b6-4831-9b12-69abc92aa4b4\"},{\"content\":{\"connectorIds\":[\"LConn3\",\"LConn4\"],\"side\":\"TOP\"},\"type\":\"ConnectorPlacement.EquallySpacedRectSide\",\"uuid\":\"2d8cca64-5216-4108-8582-3d735b4d6af0\"},{\"content\":{\"connectorIds\":[\"RConn1\"],\"side\":\"BOTTOM\"},\"type\":\"ConnectorPlacement.EquallySpacedRectSide\",\"uuid\":\"da22ed5b-3a7b-44e1-acef-3ebda742cad5\"}]},\"type\":\"ConnectorPlacement.EquallySpacedConnector\",\"uuid\":\"49f96526-0040-486f-9e93-d2a8b3aa1224\"}],\"packageUris\":[\"http://schema.mathworks.com/mf0/Connector/R2020b\"],\"version\":\"1.0\"}"
  Subsystem37 : Subsystem
      settings: PortSchema="{\"entries\":[{\"content\":{\"sides\":[{\"content\":{\"connectorIds\":[\"LConn1\",\"LConn2\"]},\"type\":\"ConnectorPlacement.EquallySpacedRectSide\",\"uuid\":\"15b6a701-c482-4ab4-b894-e969b74b8fe7\"},{\"content\":{\"side\":\"RIGHT\"},\"type\":\"ConnectorPlacement.EquallySpacedRectSide\",\"uuid\":\"d0e695dd-06b6-4831-9b12-69abc92aa4b4\"},{\"content\":{\"connectorIds\":[\"LConn3\",\"LConn4\"],\"side\":\"TOP\"},\"type\":\"ConnectorPlacement.EquallySpacedRectSide\",\"uuid\":\"2d8cca64-5216-4108-8582-3d735b4d6af0\"},{\"content\":{\"connectorIds\":[\"RConn1\"],\"side\":\"BOTTOM\"},\"type\":\"ConnectorPlacement.EquallySpacedRectSide\",\"uuid\":\"da22ed5b-3a7b-44e1-acef-3ebda742cad5\"}]},\"type\":\"ConnectorPlacement.EquallySpacedConnector\",\"uuid\":\"49f96526-0040-486f-9e93-d2a8b3aa1224\"}],\"packageUris\":[\"http://schema.mathworks.com/mf0/Connector/R2020b\"],\"version\":\"1.0\"}"
  Subsystem38 : Subsystem
      settings: PortSchema="{\"entries\":[{\"content\":{\"sides\":[{\"content\":{\"connectorIds\":[\"LConn1\",\"LConn2\"]},\"type\":\"ConnectorPlacement.EquallySpacedRectSide\",\"uuid\":\"15b6a701-c482-4ab4-b894-e969b74b8fe7\"},{\"content\":{\"side\":\"RIGHT\"},\"type\":\"ConnectorPlacement.EquallySpacedRectSide\",\"uuid\":\"d0e695dd-06b6-4831-9b12-69abc92aa4b4\"},{\"content\":{\"connectorIds\":[\"LConn3\",\"LConn4\"],\"side\":\"TOP\"},\"type\":\"ConnectorPlacement.EquallySpacedRectSide\",\"uuid\":\"2d8cca64-5216-4108-8582-3d735b4d6af0\"},{\"content\":{\"connectorIds\":[\"RConn1\"],\"side\":\"BOTTOM\"},\"type\":\"ConnectorPlacement.EquallySpacedRectSide\",\"uuid\":\"da22ed5b-3a7b-44e1-acef-3ebda742cad5\"}]},\"type\":\"ConnectorPlacement.EquallySpacedConnector\",\"uuid\":\"49f96526-0040-486f-9e93-d2a8b3aa1224\"}],\"packageUris\":[\"http://schema.mathworks.com/mf0/Connector/R2020b\"],\"version\":\"1.0\"}"
  Subsystem39 : Subsystem
      settings: PortSchema="{\"entries\":[{\"content\":{\"sides\":[{\"content\":{\"connectorIds\":[\"LConn1\",\"LConn2\"]},\"type\":\"ConnectorPlacement.EquallySpacedRectSide\",\"uuid\":\"15b6a701-c482-4ab4-b894-e969b74b8fe7\"},{\"content\":{\"side\":\"RIGHT\"},\"type\":\"ConnectorPlacement.EquallySpacedRectSide\",\"uuid\":\"d0e695dd-06b6-4831-9b12-69abc92aa4b4\"},{\"content\":{\"connectorIds\":[\"LConn3\",\"LConn4\"],\"side\":\"TOP\"},\"type\":\"ConnectorPlacement.EquallySpacedRectSide\",\"uuid\":\"2d8cca64-5216-4108-8582-3d735b4d6af0\"},{\"content\":{\"connectorIds\":[\"RConn1\"],\"side\":\"BOTTOM\"},\"type\":\"ConnectorPlacement.EquallySpacedRectSide\",\"uuid\":\"da22ed5b-3a7b-44e1-acef-3ebda742cad5\"}]},\"type\":\"ConnectorPlacement.EquallySpacedConnector\",\"uuid\":\"49f96526-0040-486f-9e93-d2a8b3aa1224\"}],\"packageUris\":[\"http://schema.mathworks.com/mf0/Connector/R2020b\"],\"version\":\"1.0\"}"
  Subsystem40 : Subsystem
      settings: PortSchema="{\"entries\":[{\"content\":{\"sides\":[{\"content\":{\"connectorIds\":[\"LConn1\",\"LConn2\"]},\"type\":\"ConnectorPlacement.EquallySpacedRectSide\",\"uuid\":\"15b6a701-c482-4ab4-b894-e969b74b8fe7\"},{\"content\":{\"side\":\"RIGHT\"},\"type\":\"ConnectorPlacement.EquallySpacedRectSide\",\"uuid\":\"d0e695dd-06b6-4831-9b12-69abc92aa4b4\"},{\"content\":{\"connectorIds\":[\"LConn3\",\"LConn4\"],\"side\":\"TOP\"},\"type\":\"ConnectorPlacement.EquallySpacedRectSide\",\"uuid\":\"2d8cca64-5216-4108-8582-3d735b4d6af0\"},{\"content\":{\"connectorIds\":[\"RConn1\"],\"side\":\"BOTTOM\"},\"type\":\"ConnectorPlacement.EquallySpacedRectSide\",\"uuid\":\"da22ed5b-3a7b-44e1-acef-3ebda742cad5\"}]},\"type\":\"ConnectorPlacement.EquallySpacedConnector\",\"uuid\":\"49f96526-0040-486f-9e93-d2a8b3aa1224\"}],\"packageUris\":[\"http://schema.mathworks.com/mf0/Connector/R2020b\"],\"version\":\"1.0\"}"
  Subsystem41 : Subsystem
      settings: PortSchema="{\"entries\":[{\"content\":{\"sides\":[{\"content\":{\"connectorIds\":[\"LConn1\",\"LConn2\"]},\"type\":\"ConnectorPlacement.EquallySpacedRectSide\",\"uuid\":\"15b6a701-c482-4ab4-b894-e969b74b8fe7\"},{\"content\":{\"side\":\"RIGHT\"},\"type\":\"ConnectorPlacement.EquallySpacedRectSide\",\"uuid\":\"d0e695dd-06b6-4831-9b12-69abc92aa4b4\"},{\"content\":{\"connectorIds\":[\"LConn3\",\"LConn4\"],\"side\":\"TOP\"},\"type\":\"ConnectorPlacement.EquallySpacedRectSide\",\"uuid\":\"2d8cca64-5216-4108-8582-3d735b4d6af0\"},{\"content\":{\"connectorIds\":[\"RConn1\"],\"side\":\"BOTTOM\"},\"type\":\"ConnectorPlacement.EquallySpacedRectSide\",\"uuid\":\"da22ed5b-3a7b-44e1-acef-3ebda742cad5\"}]},\"type\":\"ConnectorPlacement.EquallySpacedConnector\",\"uuid\":\"49f96526-0040-486f-9e93-d2a8b3aa1224\"}],\"packageUris\":[\"http://schema.mathworks.com/mf0/Connector/R2020b\"],\"version\":\"1.0\"}"
  Subsystem42 : Subsystem
      settings: PortSchema="{\"entries\":[{\"content\":{\"sides\":[{\"content\":{\"connectorIds\":[\"LConn1\",\"LConn2\"]},\"type\":\"ConnectorPlacement.EquallySpacedRectSide\",\"uuid\":\"15b6a701-c482-4ab4-b894-e969b74b8fe7\"},{\"content\":{\"side\":\"RIGHT\"},\"type\":\"ConnectorPlacement.EquallySpacedRectSide\",\"uuid\":\"d0e695dd-06b6-4831-9b12-69abc92aa4b4\"},{\"content\":{\"connectorIds\":[\"LConn3\",\"LConn4\"],\"side\":\"TOP\"},\"type\":\"ConnectorPlacement.EquallySpacedRectSide\",\"uuid\":\"2d8cca64-5216-4108-8582-3d735b4d6af0\"},{\"content\":{\"connectorIds\":[\"RConn1\"],\"side\":\"BOTTOM\"},\"type\":\"ConnectorPlacement.EquallySpacedRectSide\",\"uuid\":\"da22ed5b-3a7b-44e1-acef-3ebda742cad5\"}]},\"type\":\"ConnectorPlacement.EquallySpacedConnector\",\"uuid\":\"49f96526-0040-486f-9e93-d2a8b3aa1224\"}],\"packageUris\":[\"http://schema.mathworks.com/mf0/Connector/R2020b\"],\"version\":\"1.0\"}"
  Subsystem43 : Subsystem
      settings: PortSchema="{\"entries\":[{\"content\":{\"sides\":[{\"content\":{\"connectorIds\":[\"LConn1\",\"LConn2\"]},\"type\":\"ConnectorPlacement.EquallySpacedRectSide\",\"uuid\":\"15b6a701-c482-4ab4-b894-e969b74b8fe7\"},{\"content\":{\"side\":\"RIGHT\"},\"type\":\"ConnectorPlacement.EquallySpacedRectSide\",\"uuid\":\"d0e695dd-06b6-4831-9b12-69abc92aa4b4\"},{\"content\":{\"connectorIds\":[\"LConn3\",\"LConn4\"],\"side\":\"TOP\"},\"type\":\"ConnectorPlacement.EquallySpacedRectSide\",\"uuid\":\"2d8cca64-5216-4108-8582-3d735b4d6af0\"},{\"content\":{\"connectorIds\":[\"RConn1\"],\"side\":\"BOTTOM\"},\"type\":\"ConnectorPlacement.EquallySpacedRectSide\",\"uuid\":\"da22ed5b-3a7b-44e1-acef-3ebda742cad5\"}]},\"type\":\"ConnectorPlacement.EquallySpacedConnector\",\"uuid\":\"49f96526-0040-486f-9e93-d2a8b3aa1224\"}],\"packageUris\":[\"http://schema.mathworks.com/mf0/Connector/R2020b\"],\"version\":\"1.0\"}"
  Subsystem44 : Subsystem
      settings: PortSchema="{\"entries\":[{\"content\":{\"sides\":[{\"content\":{\"connectorIds\":[\"LConn1\",\"LConn2\"]},\"type\":\"ConnectorPlacement.EquallySpacedRectSide\",\"uuid\":\"15b6a701-c482-4ab4-b894-e969b74b8fe7\"},{\"content\":{\"side\":\"RIGHT\"},\"type\":\"ConnectorPlacement.EquallySpacedRectSide\",\"uuid\":\"d0e695dd-06b6-4831-9b12-69abc92aa4b4\"},{\"content\":{\"connectorIds\":[\"LConn3\",\"LConn4\"],\"side\":\"TOP\"},\"type\":\"ConnectorPlacement.EquallySpacedRectSide\",\"uuid\":\"2d8cca64-5216-4108-8582-3d735b4d6af0\"},{\"content\":{\"connectorIds\":[\"RConn1\"],\"side\":\"BOTTOM\"},\"type\":\"ConnectorPlacement.EquallySpacedRectSide\",\"uuid\":\"da22ed5b-3a7b-44e1-acef-3ebda742cad5\"}]},\"type\":\"ConnectorPlacement.EquallySpacedConnector\",\"uuid\":\"49f96526-0040-486f-9e93-d2a8b3aa1224\"}],\"packageUris\":[\"http://schema.mathworks.com/mf0/Connector/R2020b\"],\"version\":\"1.0\"}"
  Subsystem45 : Subsystem
      settings: PortSchema="{\"entries\":[{\"content\":{\"sides\":[{\"content\":{\"connectorIds\":[\"LConn1\",\"LConn2\"]},\"type\":\"ConnectorPlacement.EquallySpacedRectSide\",\"uuid\":\"15b6a701-c482-4ab4-b894-e969b74b8fe7\"},{\"content\":{\"side\":\"RIGHT\"},\"type\":\"ConnectorPlacement.EquallySpacedRectSide\",\"uuid\":\"d0e695dd-06b6-4831-9b12-69abc92aa4b4\"},{\"content\":{\"connectorIds\":[\"LConn3\",\"LConn4\"],\"side\":\"TOP\"},\"type\":\"ConnectorPlacement.EquallySpacedRectSide\",\"uuid\":\"2d8cca64-5216-4108-8582-3d735b4d6af0\"},{\"content\":{\"connectorIds\":[\"RConn1\"],\"side\":\"BOTTOM\"},\"type\":\"ConnectorPlacement.EquallySpacedRectSide\",\"uuid\":\"da22ed5b-3a7b-44e1-acef-3ebda742cad5\"}]},\"type\":\"ConnectorPlacement.EquallySpacedConnector\",\"uuid\":\"49f96526-0040-486f-9e93-d2a8b3aa1224\"}],\"packageUris\":[\"http://schema.mathworks.com/mf0/Connector/R2020b\"],\"version\":\"1.0\"}"
  Subsystem46 : Subsystem
      settings: PortSchema="{\"entries\":[{\"content\":{\"sides\":[{\"content\":{\"connectorIds\":[\"LConn1\",\"LConn2\"]},\"type\":\"ConnectorPlacement.EquallySpacedRectSide\",\"uuid\":\"15b6a701-c482-4ab4-b894-e969b74b8fe7\"},{\"content\":{\"side\":\"RIGHT\"},\"type\":\"ConnectorPlacement.EquallySpacedRectSide\",\"uuid\":\"d0e695dd-06b6-4831-9b12-69abc92aa4b4\"},{\"content\":{\"connectorIds\":[\"LConn3\",\"LConn4\"],\"side\":\"TOP\"},\"type\":\"ConnectorPlacement.EquallySpacedRectSide\",\"uuid\":\"2d8cca64-5216-4108-8582-3d735b4d6af0\"},{\"content\":{\"connectorIds\":[\"RConn1\"],\"side\":\"BOTTOM\"},\"type\":\"ConnectorPlacement.EquallySpacedRectSide\",\"uuid\":\"da22ed5b-3a7b-44e1-acef-3ebda742cad5\"}]},\"type\":\"ConnectorPlacement.EquallySpacedConnector\",\"uuid\":\"49f96526-0040-486f-9e93-d2a8b3aa1224\"}],\"packageUris\":[\"http://schema.mathworks.com/mf0/Connector/R2020b\"],\"version\":\"1.0\"}"
  Subsystem47 : Subsystem
      settings: PortSchema="{\"entries\":[{\"content\":{\"sides\":[{\"content\":{\"connectorIds\":[\"LConn1\",\"LConn2\"]},\"type\":\"ConnectorPlacement.EquallySpacedRectSide\",\"uuid\":\"15b6a701-c482-4ab4-b894-e969b74b8fe7\"},{\"content\":{\"side\":\"RIGHT\"},\"type\":\"ConnectorPlacement.EquallySpacedRectSide\",\"uuid\":\"d0e695dd-06b6-4831-9b12-69abc92aa4b4\"},{\"content\":{\"connectorIds\":[\"LConn3\",\"LConn4\"],\"side\":\"TOP\"},\"type\":\"ConnectorPlacement.EquallySpacedRectSide\",\"uuid\":\"2d8cca64-5216-4108-8582-3d735b4d6af0\"},{\"content\":{\"connectorIds\":[\"RConn1\"],\"side\":\"BOTTOM\"},\"type\":\"ConnectorPlacement.EquallySpacedRectSide\",\"uuid\":\"da22ed5b-3a7b-44e1-acef-3ebda742cad5\"}]},\"type\":\"ConnectorPlacement.EquallySpacedConnector\",\"uuid\":\"49f96526-0040-486f-9e93-d2a8b3aa1224\"}],\"packageUris\":[\"http://schema.mathworks.com/mf0/Connector/R2020b\"],\"version\":\"1.0\"}"
  Subsystem48 : Subsystem
      settings: PortSchema="{\"entries\":[{\"content\":{\"sides\":[{\"content\":{\"connectorIds\":[\"LConn1\",\"LConn2\"]},\"type\":\"ConnectorPlacement.EquallySpacedRectSide\",\"uuid\":\"15b6a701-c482-4ab4-b894-e969b74b8fe7\"},{\"content\":{\"side\":\"RIGHT\"},\"type\":\"ConnectorPlacement.EquallySpacedRectSide\",\"uuid\":\"d0e695dd-06b6-4831-9b12-69abc92aa4b4\"},{\"content\":{\"connectorIds\":[\"LConn3\",\"LConn4\"],\"side\":\"TOP\"},\"type\":\"ConnectorPlacement.EquallySpacedRectSide\",\"uuid\":\"2d8cca64-5216-4108-8582-3d735b4d6af0\"},{\"content\":{\"connectorIds\":[\"RConn1\"],\"side\":\"BOTTOM\"},\"type\":\"ConnectorPlacement.EquallySpacedRectSide\",\"uuid\":\"da22ed5b-3a7b-44e1-acef-3ebda742cad5\"}]},\"type\":\"ConnectorPlacement.EquallySpacedConnector\",\"uuid\":\"49f96526-0040-486f-9e93-d2a8b3aa1224\"}],\"packageUris\":[\"http://schema.mathworks.com/mf0/Connector/R2020b\"],\"version\":\"1.0\"}"
  Subsystem49 : Subsystem
      settings: PortSchema="{\"entries\":[{\"content\":{\"sides\":[{\"content\":{\"connectorIds\":[\"LConn1\",\"LConn2\"]},\"type\":\"ConnectorPlacement.EquallySpacedRectSide\",\"uuid\":\"15b6a701-c482-4ab4-b894-e969b74b8fe7\"},{\"content\":{\"side\":\"RIGHT\"},\"type\":\"ConnectorPlacement.EquallySpacedRectSide\",\"uuid\":\"d0e695dd-06b6-4831-9b12-69abc92aa4b4\"},{\"content\":{\"connectorIds\":[\"LConn3\",\"LConn4\"],\"side\":\"TOP\"},\"type\":\"ConnectorPlacement.EquallySpacedRectSide\",\"uuid\":\"2d8cca64-5216-4108-8582-3d735b4d6af0\"},{\"content\":{\"connectorIds\":[\"RConn1\"],\"side\":\"BOTTOM\"},\"type\":\"ConnectorPlacement.EquallySpacedRectSide\",\"uuid\":\"da22ed5b-3a7b-44e1-acef-3ebda742cad5\"}]},\"type\":\"ConnectorPlacement.EquallySpacedConnector\",\"uuid\":\"49f96526-0040-486f-9e93-d2a8b3aa1224\"}],\"packageUris\":[\"http://schema.mathworks.com/mf0/Connector/R2020b\"],\"version\":\"1.0\"}"
  Subsystem51 : Subsystem
      settings: PortSchema="{\"entries\":[{\"content\":{\"sides\":[{\"content\":{\"connectorIds\":[\"LConn1\",\"LConn2\"]},\"type\":\"ConnectorPlacement.EquallySpacedRectSide\",\"uuid\":\"15b6a701-c482-4ab4-b894-e969b74b8fe7\"},{\"content\":{\"side\":\"RIGHT\"},\"type\":\"ConnectorPlacement.EquallySpacedRectSide\",\"uuid\":\"d0e695dd-06b6-4831-9b12-69abc92aa4b4\"},{\"content\":{\"connectorIds\":[\"LConn3\",\"LConn4\"],\"side\":\"TOP\"},\"type\":\"ConnectorPlacement.EquallySpacedRectSide\",\"uuid\":\"2d8cca64-5216-4108-8582-3d735b4d6af0\"},{\"content\":{\"connectorIds\":[\"RConn1\"],\"side\":\"BOTTOM\"},\"type\":\"ConnectorPlacement.EquallySpacedRectSide\",\"uuid\":\"da22ed5b-3a7b-44e1-acef-3ebda742cad5\"}]},\"type\":\"ConnectorPlacement.EquallySpacedConnector\",\"uuid\":\"49f96526-0040-486f-9e93-d2a8b3aa1224\"}],\"packageUris\":[\"http://schema.mathworks.com/mf0/Connector/R2020b\"],\"version\":\"1.0\"}"
  Subsystem52 : Subsystem
      settings: PortSchema="{\"entries\":[{\"content\":{\"sides\":[{\"content\":{\"connectorIds\":[\"LConn1\",\"LConn2\"]},\"type\":\"ConnectorPlacement.EquallySpacedRectSide\",\"uuid\":\"15b6a701-c482-4ab4-b894-e969b74b8fe7\"},{\"content\":{\"side\":\"RIGHT\"},\"type\":\"ConnectorPlacement.EquallySpacedRectSide\",\"uuid\":\"d0e695dd-06b6-4831-9b12-69abc92aa4b4\"},{\"content\":{\"connectorIds\":[\"LConn3\",\"LConn4\"],\"side\":\"TOP\"},\"type\":\"ConnectorPlacement.EquallySpacedRectSide\",\"uuid\":\"2d8cca64-5216-4108-8582-3d735b4d6af0\"},{\"content\":{\"connectorIds\":[\"RConn1\"],\"side\":\"BOTTOM\"},\"type\":\"ConnectorPlacement.EquallySpacedRectSide\",\"uuid\":\"da22ed5b-3a7b-44e1-acef-3ebda742cad5\"}]},\"type\":\"ConnectorPlacement.EquallySpacedConnector\",\"uuid\":\"49f96526-0040-486f-9e93-d2a8b3aa1224\"}],\"packageUris\":[\"http://schema.mathworks.com/mf0/Connector/R2020b\"],\"version\":\"1.0\"}"
  Subsystem53 : Subsystem
      settings: PortSchema="{\"entries\":[{\"content\":{\"sides\":[{\"content\":{\"connectorIds\":[\"LConn1\",\"LConn2\"]},\"type\":\"ConnectorPlacement.EquallySpacedRectSide\",\"uuid\":\"15b6a701-c482-4ab4-b894-e969b74b8fe7\"},{\"content\":{\"side\":\"RIGHT\"},\"type\":\"ConnectorPlacement.EquallySpacedRectSide\",\"uuid\":\"d0e695dd-06b6-4831-9b12-69abc92aa4b4\"},{\"content\":{\"connectorIds\":[\"LConn3\",\"LConn4\"],\"side\":\"TOP\"},\"type\":\"ConnectorPlacement.EquallySpacedRectSide\",\"uuid\":\"2d8cca64-5216-4108-8582-3d735b4d6af0\"},{\"content\":{\"connectorIds\":[\"RConn1\"],\"side\":\"BOTTOM\"},\"type\":\"ConnectorPlacement.EquallySpacedRectSide\",\"uuid\":\"da22ed5b-3a7b-44e1-acef-3ebda742cad5\"}]},\"type\":\"ConnectorPlacement.EquallySpacedConnector\",\"uuid\":\"49f96526-0040-486f-9e93-d2a8b3aa1224\"}],\"packageUris\":[\"http://schema.mathworks.com/mf0/Connector/R2020b\"],\"version\":\"1.0\"}"
  Subsystem54 : Subsystem
      settings: PortSchema="{\"entries\":[{\"content\":{\"sides\":[{\"content\":{\"connectorIds\":[\"LConn1\",\"LConn2\"]},\"type\":\"ConnectorPlacement.EquallySpacedRectSide\",\"uuid\":\"15b6a701-c482-4ab4-b894-e969b74b8fe7\"},{\"content\":{\"side\":\"RIGHT\"},\"type\":\"ConnectorPlacement.EquallySpacedRectSide\",\"uuid\":\"d0e695dd-06b6-4831-9b12-69abc92aa4b4\"},{\"content\":{\"connectorIds\":[\"LConn3\",\"LConn4\"],\"side\":\"TOP\"},\"type\":\"ConnectorPlacement.EquallySpacedRectSide\",\"uuid\":\"2d8cca64-5216-4108-8582-3d735b4d6af0\"},{\"content\":{\"connectorIds\":[\"RConn1\"],\"side\":\"BOTTOM\"},\"type\":\"ConnectorPlacement.EquallySpacedRectSide\",\"uuid\":\"da22ed5b-3a7b-44e1-acef-3ebda742cad5\"}]},\"type\":\"ConnectorPlacement.EquallySpacedConnector\",\"uuid\":\"49f96526-0040-486f-9e93-d2a8b3aa1224\"}],\"packageUris\":[\"http://schema.mathworks.com/mf0/Connector/R2020b\"],\"version\":\"1.0\"}"
  Subsystem6 : Subsystem
      settings: PortSchema="{\"entries\":[{\"content\":{\"sides\":[{\"content\":{\"connectorIds\":[\"LConn1\",\"LConn2\"]},\"type\":\"ConnectorPlacement.EquallySpacedRectSide\",\"uuid\":\"15b6a701-c482-4ab4-b894-e969b74b8fe7\"},{\"content\":{\"side\":\"RIGHT\"},\"type\":\"ConnectorPlacement.EquallySpacedRectSide\",\"uuid\":\"d0e695dd-06b6-4831-9b12-69abc92aa4b4\"},{\"content\":{\"connectorIds\":[\"LConn3\",\"LConn4\"],\"side\":\"TOP\"},\"type\":\"ConnectorPlacement.EquallySpacedRectSide\",\"uuid\":\"2d8cca64-5216-4108-8582-3d735b4d6af0\"},{\"content\":{\"connectorIds\":[\"RConn1\"],\"side\":\"BOTTOM\"},\"type\":\"ConnectorPlacement.EquallySpacedRectSide\",\"uuid\":\"da22ed5b-3a7b-44e1-acef-3ebda742cad5\"}]},\"type\":\"ConnectorPlacement.EquallySpacedConnector\",\"uuid\":\"49f96526-0040-486f-9e93-d2a8b3aa1224\"}],\"packageUris\":[\"http://schema.mathworks.com/mf0/Connector/R2020b\"],\"version\":\"1.0\"}"
  Subsystem7 : Subsystem
      settings: PortSchema="{\"entries\":[{\"content\":{\"sides\":[{\"content\":{\"connectorIds\":[\"LConn1\",\"LConn2\"]},\"type\":\"ConnectorPlacement.EquallySpacedRectSide\",\"uuid\":\"15b6a701-c482-4ab4-b894-e969b74b8fe7\"},{\"content\":{\"side\":\"RIGHT\"},\"type\":\"ConnectorPlacement.EquallySpacedRectSide\",\"uuid\":\"d0e695dd-06b6-4831-9b12-69abc92aa4b4\"},{\"content\":{\"connectorIds\":[\"LConn3\",\"LConn4\"],\"side\":\"TOP\"},\"type\":\"ConnectorPlacement.EquallySpacedRectSide\",\"uuid\":\"2d8cca64-5216-4108-8582-3d735b4d6af0\"},{\"content\":{\"connectorIds\":[\"RConn1\"],\"side\":\"BOTTOM\"},\"type\":\"ConnectorPlacement.EquallySpacedRectSide\",\"uuid\":\"da22ed5b-3a7b-44e1-acef-3ebda742cad5\"}]},\"type\":\"ConnectorPlacement.EquallySpacedConnector\",\"uuid\":\"49f96526-0040-486f-9e93-d2a8b3aa1224\"}],\"packageUris\":[\"http://schema.mathworks.com/mf0/Connector/R2020b\"],\"version\":\"1.0\"}"
  Subsystem8 : Subsystem
      settings: PortSchema="{\"entries\":[{\"content\":{\"sides\":[{\"content\":{\"connectorIds\":[\"LConn1\",\"LConn2\"]},\"type\":\"ConnectorPlacement.EquallySpacedRectSide\",\"uuid\":\"15b6a701-c482-4ab4-b894-e969b74b8fe7\"},{\"content\":{\"side\":\"RIGHT\"},\"type\":\"ConnectorPlacement.EquallySpacedRectSide\",\"uuid\":\"d0e695dd-06b6-4831-9b12-69abc92aa4b4\"},{\"content\":{\"connectorIds\":[\"LConn3\",\"LConn4\"],\"side\":\"TOP\"},\"type\":\"ConnectorPlacement.EquallySpacedRectSide\",\"uuid\":\"2d8cca64-5216-4108-8582-3d735b4d6af0\"},{\"content\":{\"connectorIds\":[\"RConn1\"],\"side\":\"BOTTOM\"},\"type\":\"ConnectorPlacement.EquallySpacedRectSide\",\"uuid\":\"da22ed5b-3a7b-44e1-acef-3ebda742cad5\"}]},\"type\":\"ConnectorPlacement.EquallySpacedConnector\",\"uuid\":\"49f96526-0040-486f-9e93-d2a8b3aa1224\"}],\"packageUris\":[\"http://schema.mathworks.com/mf0/Connector/R2020b\"],\"version\":\"1.0\"}"
  Subsystem9 : Subsystem
      settings: PortSchema="{\"entries\":[{\"content\":{\"sides\":[{\"content\":{\"connectorIds\":[\"LConn1\",\"LConn2\"]},\"type\":\"ConnectorPlacement.EquallySpacedRectSide\",\"uuid\":\"15b6a701-c482-4ab4-b894-e969b74b8fe7\"},{\"content\":{\"side\":\"RIGHT\"},\"type\":\"ConnectorPlacement.EquallySpacedRectSide\",\"uuid\":\"d0e695dd-06b6-4831-9b12-69abc92aa4b4\"},{\"content\":{\"connectorIds\":[\"LConn3\",\"LConn4\"],\"side\":\"TOP\"},\"type\":\"ConnectorPlacement.EquallySpacedRectSide\",\"uuid\":\"2d8cca64-5216-4108-8582-3d735b4d6af0\"},{\"content\":{\"connectorIds\":[\"RConn1\"],\"side\":\"BOTTOM\"},\"type\":\"ConnectorPlacement.EquallySpacedRectSide\",\"uuid\":\"da22ed5b-3a7b-44e1-acef-3ebda742cad5\"}]},\"type\":\"ConnectorPlacement.EquallySpacedConnector\",\"uuid\":\"49f96526-0040-486f-9e93-d2a8b3aa1224\"}],\"packageUris\":[\"http://schema.mathworks.com/mf0/Connector/R2020b\"],\"version\":\"1.0\"}"
  Sum : Sum  Inputs=|++
  Sum1 : Sum  Inputs=+-
  Unit Delay{,1..3} (4 alike) : UnitDelay  SampleTime=-1
  Voltage Source : ee_lib/Sources/Voltage Source  dc_voltage=375.5 V  ac_voltage=0 V  ac_shift=0 rad  ac_frequency=60 Hz  noise_mode=ee.enum.sources.noise.Disabled  PSD=0 V^2/Hz  sample_time=1e-3 s  repeatability=ee.enum.sources.repeatability.NotRepeatable  user_seed=0  auto_seed=3499211588  i_specify=off  i_priority=None  i=0 A  i_nominal_specify=off  i_nominal_value=1  i_nominal_unit=A  v_specify=off  v_priority=None  v=0 V  v_nominal_specify=off  v_nominal_value=1  v_nominal_unit=V
  Voltage Source1 : ee_lib/Sources/Voltage Source  dc_voltage=375.5 V  ac_voltage=0 V  ac_shift=0 rad  ac_frequency=60 Hz  noise_mode=ee.enum.sources.noise.Disabled  PSD=0 V^2/Hz  sample_time=1e-3 s  repeatability=ee.enum.sources.repeatability.NotRepeatable  user_seed=0  auto_seed=2915145293  i_specify=off  i_priority=None  i=0 A  i_nominal_specify=off  i_nominal_value=1  i_nominal_unit=A  v_specify=off  v_priority=None  v=0 V  v_nominal_specify=off  v_nominal_value=1  v_nominal_unit=V
  ia_ref : Sin  Frequency=2*pi*50  SampleTime=0
  tag scope: ia_circ=global, ia_lower=global, ia_meas=global, ia_upper=global, ib_lower=global, ib_meas=global, ib_upper=global, ic_lower=global, ic_meas=global, ic_upper=global, la_SM1_Vc=global, la_SM2_Vc=global, la_SM3_Vc=global, la_SM4_Vc=global, la_SM5_Vc=global, la_SM6_Vc=global, la_SM7_Vc=global, la_SM8_Vc=global, lb_SM1_Vc=global, lb_SM2_Vc=global, lb_SM3_Vc=global, lb_SM4_Vc=global, lb_SM5_Vc=global, lb_SM6_Vc=global, lb_SM7_Vc=global, lb_SM8_Vc=global, lc_SM1_Vc=global, lc_SM2_Vc=global, lc_SM3_Vc=global, lc_SM4_Vc=global, lc_SM5_Vc=global, lc_SM6_Vc=global, lc_SM7_Vc=global, lc_SM8_Vc=global, ua_SM1_Vc=global, ua_SM2_Vc=global, ua_SM3_Vc=global, ua_SM4_Vc=global, ua_SM5_Vc=global, ua_SM6_Vc=global, ua_SM7_Vc=global, ua_SM8_Vc=global, ub_SM1_Vc=global, ub_SM2_Vc=global, ub_SM3_Vc=global, ub_SM4_Vc=global, ub_SM5_Vc=global, ub_SM6_Vc=global, ub_SM7_Vc=global, ub_SM8_Vc=global, uc_SM1_Vc=global, uc_SM2_Vc=global, uc_SM3_Vc=global, uc_SM4_Vc=global, uc_SM5_Vc=global, uc_SM6_Vc=global, uc_SM7_Vc=global, uc_SM8_Vc=global
  wires:
  PS-Simulink Converter10/1 -> [I_dc]  "I_dc"
  PS-Simulink Converter4/1 -> [ia_lower]  "ia_lower"
  PS-Simulink Converter5/1 -> [ib_lower]  "ib_lower"
  PS-Simulink Converter6/1 -> [ic_lower]  "ic_lower"
  PS-Simulink Converter1/1 -> [ia_upper]  "ia_upper"
  PS-Simulink Converter2/1 -> [ib_upper]  "ib_upper"
  PS-Simulink Converter3/1 -> [ic_upper]  "ic_upper"
  PS-Simulink Converter8/1 -> [ia_meas]  "i_a"
  PS-Simulink Converter7/1 -> [ib_meas]  "i_b"
  PS-Simulink Converter9/1 -> [ic_meas]  "i_c"
  Constant/1 -> MATLAB Function1/8(Vdc)
  ia_ref/1 -> MATLAB Function1/1(i_ref)
  Rarm/1 -> MATLAB Function1/15(Rarm)
  Constant1/1 -> MATLAB Function1/10(N)
  Constant2/1 -> MATLAB Function1/16(L_load)
  Constant3/1 -> MATLAB Function1/17(R_load)
  [ia_meas] -> MATLAB Function1/2(i_out_meas)
  [ia_upper] -> MATLAB Function1/4(i_upper)
  [ia_lower] -> MATLAB Function1/5(i_lower)
  [ia_upper] -> Sum/1
  [ia_lower] -> Sum/2
  Sum/1 -> Gain/1
  Gain/1 -> Sum1/1
  [I_dc] -> Gain1/1
  Gain1/1 -> Sum1/2
  Sum1/1 -> [ia_circ]  "ia_circ"
  [ia_circ] -> MATLAB Function1/3(i_circ_meas)
  PS-Simulink Converter/1 -> [ua_SM1_Vc]
  PS-Simulink Converter11/1 -> [ua_SM2_Vc]
  PS-Simulink Converter12/1 -> [ua_SM3_Vc]
  PS-Simulink Converter13/1 -> [ua_SM4_Vc]
  PS-Simulink Converter14/1 -> [ua_SM5_Vc]
  PS-Simulink Converter15/1 -> [ua_SM6_Vc]
  PS-Simulink Converter16/1 -> [ua_SM7_Vc]
  PS-Simulink Converter17/1 -> [ua_SM8_Vc]
  PS-Simulink Converter18/1 -> [ub_SM8_Vc]
  PS-Simulink Converter19/1 -> [uc_SM8_Vc]
  PS-Simulink Converter20/1 -> [ub_SM7_Vc]
  PS-Simulink Converter21/1 -> [uc_SM7_Vc]
  PS-Simulink Converter22/1 -> [ub_SM6_Vc]
  PS-Simulink Converter23/1 -> [uc_SM6_Vc]
  PS-Simulink Converter24/1 -> [ub_SM5_Vc]
  PS-Simulink Converter25/1 -> [uc_SM5_Vc]
  PS-Simulink Converter26/1 -> [ub_SM4_Vc]
  PS-Simulink Converter27/1 -> [uc_SM4_Vc]
  PS-Simulink Converter28/1 -> [ub_SM3_Vc]
  PS-Simulink Converter29/1 -> [uc_SM3_Vc]
  PS-Simulink Converter30/1 -> [ub_SM2_Vc]
  PS-Simulink Converter31/1 -> [uc_SM2_Vc]
  PS-Simulink Converter32/1 -> [ub_SM1_Vc]
  PS-Simulink Converter33/1 -> [uc_SM1_Vc]
  PS-Simulink Converter34/1 -> [la_SM1_Vc]
  PS-Simulink Converter35/1 -> [lb_SM1_Vc]
  PS-Simulink Converter36/1 -> [lc_SM1_Vc]
  PS-Simulink Converter37/1 -> [la_SM2_Vc]
  PS-Simulink Converter38/1 -> [lb_SM2_Vc]
  PS-Simulink Converter39/1 -> [lc_SM2_Vc]
  PS-Simulink Converter40/1 -> [la_SM3_Vc]
  PS-Simulink Converter41/1 -> [lb_SM3_Vc]
  PS-Simulink Converter42/1 -> [lc_SM3_Vc]
  PS-Simulink Converter43/1 -> [la_SM4_Vc]
  PS-Simulink Converter44/1 -> [lb_SM4_Vc]
  PS-Simulink Converter45/1 -> [lc_SM4_Vc]
  PS-Simulink Converter46/1 -> [la_SM5_Vc]
  PS-Simulink Converter47/1 -> [lb_SM5_Vc]
  PS-Simulink Converter48/1 -> [lc_SM5_Vc]
  PS-Simulink Converter49/1 -> [la_SM6_Vc]
  PS-Simulink Converter50/1 -> [lb_SM6_Vc]
  PS-Simulink Converter51/1 -> [lc_SM6_Vc]
  PS-Simulink Converter52/1 -> [la_SM7_Vc]
  PS-Simulink Converter53/1 -> [lb_SM7_Vc]
  PS-Simulink Converter54/1 -> [lc_SM7_Vc]
  PS-Simulink Converter55/1 -> [la_SM8_Vc]
  PS-Simulink Converter56/1 -> [lb_SM8_Vc]
  PS-Simulink Converter57/1 -> [lc_SM8_Vc]
  [la_SM1_Vc] -> Mux/1
  [la_SM4_Vc] -> Mux/4
  [la_SM3_Vc] -> Mux/3
  [la_SM2_Vc] -> Mux/2
  [lc_SM8_Vc] -> Mux/8
  [la_SM7_Vc] -> Mux/7
  [la_SM6_Vc] -> Mux/6
  [la_SM5_Vc] -> Mux/5
  Mux/1 -> [vcl_a]  "vcl_a"
  [vcu_a] -> MATLAB Function1/6(vcu)
  Mux1/1 -> [vcu_a]  "vcu_a"
  [ua_SM3_Vc] -> Mux1/3
  [ua_SM8_Vc] -> Mux1/8
  [ua_SM6_Vc] -> Mux1/6
  [ua_SM1_Vc] -> Mux1/1
  [ua_SM7_Vc] -> Mux1/7
  [ua_SM5_Vc] -> Mux1/5
  [ua_SM4_Vc] -> Mux1/4
  [ua_SM2_Vc] -> Mux1/2
  [vcl_a] -> MATLAB Function1/7(vcl)
  MATLAB Function1/1(nu_opt) -> [nu_opt_a], Unit Delay1/1  "nu_opt"
  Unit Delay1/1 -> [nu_prev_a]
  MATLAB Function1/2(nl_opt) -> [nl_opt_a], Unit Delay2/1  "nl_opt"
  Unit Delay2/1 -> [nl_prev_a]
  [nu_prev_a] -> MATLAB Function1/12(nu_prev)
  [nl_prev_a] -> MATLAB Function1/13(nl_prev)
  Constant4/1 -> MATLAB Function1/11(Csm)
  Constant5/1 -> MATLAB Function1/14(Larm)
  Constant6/1 -> MATLAB Function1/9(Ts)
  Constant7/1 -> MATLAB Function1/18(lambda_i)
  Constant8/1 -> MATLAB Function1/19(lambda_sw)
  Constant9/1 -> MATLAB Function1/20(lambda_cap)
  Constant10/1 -> MATLAB Function1/21(lambda_circ)
  [vcu_a] -> MATLAB Function2/1(vcu)
  [vcl_a] -> MATLAB Function2/2(vcl)
  [nu_opt_a] -> MATLAB Function2/3(nu)
  [nl_opt_a] -> MATLAB Function2/4(nl)
  [ia_upper] -> MATLAB Function2/5(i_upper)
  [ia_lower] -> MATLAB Function2/6(i_lower)
  Constant11/1 -> MATLAB Function2/9(N)
  MATLAB Function2/5(Su) -> Unit Delay/1
  MATLAB Function2/6(Sl) -> Unit Delay3/1
  Unit Delay/1 -> [Su_prev_a]
  Unit Delay3/1 -> [Sl_prev_a]
  [Su_prev_a] -> MATLAB Function2/7(Su_prev)
  [Sl_prev_a] -> MATLAB Function2/8(Sl_prev)
  connections:
  Inductor7/RConn1 -- Subsystem8/LConn3
  Resistor/RConn1 -- Electrical Reference1/LConn1 -- Resistor1/RConn1 -- Resistor2/RConn1
  Simulink-PS Converter73/RConn1 -- Subsystem48/LConn1
  Simulink-PS Converter80/RConn1 -- Subsystem48/LConn2
  Current Sensor9/RConn2 -- Subsystem48/LConn3 -- Subsystem45/LConn3 -- Subsystem21/LConn3
  Voltage Source1/RConn1 -- Subsystem1/RConn1 -- Subsystem14/RConn1 -- Subsystem35/RConn1 -- Solver Configuration1/RConn1
  Voltage Source1/LConn1 -- Electrical Reference/LConn1 -- Voltage Source/RConn1
  Subsystem7/LConn3 -- Subsystem47/RConn1
  Subsystem54/LConn3 -- Subsystem38/RConn1
  Subsystem38/LConn3 -- Subsystem48/RConn1
  Current Sensor/RConn2 -- Subsystem13/RConn1
  Subsystem16/LConn3 -- Current Sensor/LConn1
  Subsystem8/RConn1 -- Current Sensor3/RConn2
  Inductor6/RConn1 -- Inductor7/LConn1 -- Current Sensor6/LConn1
  Current Sensor8/LConn1 -- Inductor2/LConn1 -- Inductor1/RConn1
  Inductor1/LConn1 -- Subsystem9/RConn1
  Inductor2/RConn1 -- Subsystem34/LConn3
  Current Sensor7/LConn1 -- Inductor4/LConn1 -- Inductor3/RConn1
  Inductor3/LConn1 -- Subsystem33/RConn1
  Inductor4/RConn1 -- Subsystem53/LConn3
  Inductor9/LConn1 -- Resistor/LConn1
  Inductor5/RConn1 -- Current Sensor7/RConn2
  Current Sensor8/RConn1 -- PS-Simulink Converter7/LConn1
  Current Sensor6/RConn1 -- PS-Simulink Converter8/LConn1
  Current Sensor7/RConn1 -- PS-Simulink Converter9/LConn1
  Voltage Source/LConn1 -- Current Sensor9/LConn1
  Current Sensor9/RConn1 -- PS-Simulink Converter10/LConn1
  Subsystem11/LConn3 -- Current Sensor3/LConn1
  Simulink-PS Converter95/RConn1 -- Subsystem38/LConn2
  Simulink-PS Converter87/RConn1 -- Subsystem38/LConn1
  Simulink-PS Converter107/RConn1 -- Subsystem47/LConn2
  Simulink-PS Converter103/RConn1 -- Subsystem47/LConn1
  Simulink-PS Converter90/RConn1 -- Subsystem54/LConn2
  Simulink-PS Converter82/RConn1 -- Subsystem54/LConn1
  Subsystem47/LConn3 -- Subsystem54/RConn1
  Simulink-PS Converter46/RConn1 -- Subsystem37/LConn1
  Simulink-PS Converter37/RConn1 -- Subsystem13/LConn1
  Subsystem37/LConn3 -- Subsystem7/RConn1
  Subsystem13/LConn3 -- Subsystem37/RConn1
  Simulink-PS Converter44/RConn1 -- Subsystem13/LConn2
  Simulink-PS Converter92/RConn1 -- Subsystem37/LConn2
  Simulink-PS Converter47/RConn1 -- Subsystem7/LConn1
  Simulink-PS Converter93/RConn1 -- Subsystem7/LConn2
  Simulink-PS Converter8/RConn1 -- Subsystem16/LConn2
  Simulink-PS Converter7/RConn1 -- Subsystem16/LConn1
  Simulink-PS Converter50/RConn1 -- Subsystem18/LConn2
  Subsystem20/LConn3 -- Subsystem23/RConn1
  Simulink-PS Converter19/RConn1 -- Subsystem3/LConn1
  Subsystem3/LConn3 -- Subsystem18/RConn1
  Subsystem9/LConn3 -- Current Sensor1/LConn1
  Simulink-PS Converter12/RConn1 -- Subsystem20/LConn2
  Simulink-PS Converter41/RConn1 -- Subsystem9/LConn2
  Subsystem23/LConn3 -- Subsystem19/RConn1
  Simulink-PS Converter48/RConn1 -- Subsystem23/LConn2
  Simulink-PS Converter43/RConn1 -- Subsystem23/LConn1
  Simulink-PS Converter38/RConn1 -- Subsystem9/LConn1
  Simulink-PS Converter11/RConn1 -- Subsystem20/LConn1
  Subsystem19/LConn3 -- Subsystem21/RConn1
  Simulink-PS Converter21/RConn1 -- Subsystem3/LConn2
  Subsystem27/LConn3 -- Subsystem20/RConn1
  Simulink-PS Converter22/RConn1 -- Subsystem18/LConn1
  Simulink-PS Converter52/RConn1 -- Subsystem19/LConn2
  Simulink-PS Converter51/RConn1 -- Subsystem27/LConn2
  Current Sensor1/RConn2 -- Subsystem3/RConn1
  Simulink-PS Converter45/RConn1 -- Subsystem19/LConn1
  Simulink-PS Converter42/RConn1 -- Subsystem21/LConn2
  Subsystem18/LConn3 -- Subsystem27/RConn1
  Simulink-PS Converter23/RConn1 -- Subsystem27/LConn1
  Simulink-PS Converter40/RConn1 -- Subsystem21/LConn1
  Simulink-PS Converter104/RConn1 -- Subsystem42/LConn2
  Subsystem44/LConn3 -- Subsystem49/RConn1
  Simulink-PS Converter70/RConn1 -- Subsystem30/LConn1
  Subsystem30/LConn3 -- Subsystem42/RConn1
  Subsystem33/LConn3 -- Current Sensor4/LConn1
  Simulink-PS Converter59/RConn1 -- Subsystem44/LConn2
  Simulink-PS Converter96/RConn1 -- Subsystem33/LConn2
  Subsystem49/LConn3 -- Subsystem43/RConn1
  Simulink-PS Converter102/RConn1 -- Subsystem49/LConn2
  Simulink-PS Converter99/RConn1 -- Subsystem49/LConn1
  Simulink-PS Converter89/RConn1 -- Subsystem33/LConn1
  Simulink-PS Converter57/RConn1 -- Subsystem44/LConn1
  Subsystem43/LConn3 -- Subsystem45/RConn1
  Simulink-PS Converter74/RConn1 -- Subsystem30/LConn2
  Subsystem52/LConn3 -- Subsystem44/RConn1
  Simulink-PS Converter75/RConn1 -- Subsystem42/LConn1
  Simulink-PS Converter106/RConn1 -- Subsystem43/LConn2
  Simulink-PS Converter105/RConn1 -- Subsystem52/LConn2
  Current Sensor4/RConn2 -- Subsystem30/RConn1
  Simulink-PS Converter100/RConn1 -- Subsystem43/LConn1
  Simulink-PS Converter98/RConn1 -- Subsystem45/LConn2
  Subsystem42/LConn3 -- Subsystem52/RConn1
  Simulink-PS Converter76/RConn1 -- Subsystem52/LConn1
  Simulink-PS Converter94/RConn1 -- Subsystem45/LConn1
  Simulink-PS Converter3/RConn1 -- Subsystem8/LConn1
  Simulink-PS Converter4/RConn1 -- Subsystem8/LConn2
  Simulink-PS Converter10/RConn1 -- Subsystem10/LConn1
  Simulink-PS Converter28/RConn1 -- Subsystem12/LConn1
  Subsystem12/LConn3 -- Subsystem6/RConn1
  Subsystem6/LConn3 -- Subsystem11/RConn1
  Subsystem17/LConn3 -- Subsystem10/RConn1
  Simulink-PS Converter14/RConn1 -- Subsystem10/LConn2
  Simulink-PS Converter31/RConn1 -- Subsystem12/LConn2
  Simulink-PS Converter32/RConn1 -- Subsystem2/LConn2
  Subsystem10/LConn3 -- Subsystem12/RConn1
  Simulink-PS Converter17/RConn1 -- Subsystem1/LConn2
  Simulink-PS Converter24/RConn1 -- Subsystem17/LConn1
  Simulink-PS Converter33/RConn1 -- Subsystem17/LConn2
  Simulink-PS Converter34/RConn1 -- Subsystem6/LConn2
  Simulink-PS Converter30/RConn1 -- Subsystem6/LConn1
  Simulink-PS Converter16/RConn1 -- Subsystem1/LConn1
  Subsystem2/LConn3 -- Subsystem17/RConn1
  Simulink-PS Converter27/RConn1 -- Subsystem11/LConn2
  Simulink-PS Converter18/RConn1 -- Subsystem2/LConn1
  Subsystem1/LConn3 -- Subsystem2/RConn1
  Simulink-PS Converter25/RConn1 -- Subsystem11/LConn1
  Subsystem14/LConn3 -- Subsystem28/RConn1
  Simulink-PS Converter56/RConn1 -- Subsystem34/LConn1
  Simulink-PS Converter35/RConn1 -- Subsystem14/LConn2
  Simulink-PS Converter63/RConn1 -- Subsystem31/LConn2
  Simulink-PS Converter53/RConn1 -- Subsystem24/LConn1
  Simulink-PS Converter62/RConn1 -- Subsystem26/LConn2
  Subsystem34/RConn1 -- Current Sensor2/RConn2
  Simulink-PS Converter60/RConn1 -- Subsystem25/LConn2
  Simulink-PS Converter20/RConn1 -- Subsystem14/LConn1
  Simulink-PS Converter58/RConn1 -- Subsystem31/LConn1
  Subsystem28/LConn3 -- Subsystem26/RConn1
  Simulink-PS Converter13/RConn1 -- Subsystem22/LConn1
  Subsystem22/LConn3 -- Subsystem25/RConn1
  Simulink-PS Converter15/RConn1 -- Subsystem22/LConn2
  Subsystem25/LConn3 -- Subsystem31/RConn1
  Simulink-PS Converter64/RConn1 -- Subsystem34/LConn2
  Simulink-PS Converter61/RConn1 -- Subsystem28/LConn2
  Subsystem26/LConn3 -- Subsystem22/RConn1
  Simulink-PS Converter54/RConn1 -- Subsystem24/LConn2
  Simulink-PS Converter55/RConn1 -- Subsystem25/LConn1
  Simulink-PS Converter36/RConn1 -- Subsystem28/LConn1
  Subsystem31/LConn3 -- Subsystem24/RConn1
  Simulink-PS Converter49/RConn1 -- Subsystem26/LConn1
  Subsystem24/LConn3 -- Current Sensor2/LConn1
  Subsystem35/LConn3 -- Subsystem46/RConn1
  Simulink-PS Converter85/RConn1 -- Subsystem53/LConn1
  Simulink-PS Converter69/RConn1 -- Subsystem35/LConn2
  Simulink-PS Converter101/RConn1 -- Subsystem51/LConn2
  Simulink-PS Converter79/RConn1 -- Subsystem39/LConn1
  Simulink-PS Converter97/RConn1 -- Subsystem41/LConn2
  Current Sensor5/RConn2 -- Subsystem53/RConn1
  Simulink-PS Converter88/RConn1 -- Subsystem40/LConn2
  Simulink-PS Converter68/RConn1 -- Subsystem35/LConn1
  Simulink-PS Converter86/RConn1 -- Subsystem51/LConn1
  Subsystem46/LConn3 -- Subsystem41/RConn1
  Simulink-PS Converter66/RConn1 -- Subsystem36/LConn1
  Subsystem36/LConn3 -- Subsystem40/RConn1
  Simulink-PS Converter67/RConn1 -- Subsystem36/LConn2
  Subsystem40/LConn3 -- Subsystem51/RConn1
  Simulink-PS Converter108/RConn1 -- Subsystem53/LConn2
  Simulink-PS Converter91/RConn1 -- Subsystem46/LConn2
  Subsystem41/LConn3 -- Subsystem36/RConn1
  Simulink-PS Converter81/RConn1 -- Subsystem39/LConn2
  Simulink-PS Converter84/RConn1 -- Subsystem40/LConn1
  Simulink-PS Converter71/RConn1 -- Subsystem46/LConn1
  Subsystem51/LConn3 -- Subsystem39/RConn1
  Simulink-PS Converter77/RConn1 -- Subsystem41/LConn1
  Subsystem39/LConn3 -- Current Sensor5/LConn1
  PS-Simulink Converter1/LConn1 -- Current Sensor/RConn1
  Current Sensor1/RConn1 -- PS-Simulink Converter2/LConn1
  PS-Simulink Converter3/LConn1 -- Current Sensor4/RConn1
  PS-Simulink Converter4/LConn1 -- Current Sensor3/RConn1
  PS-Simulink Converter5/LConn1 -- Current Sensor2/RConn1
  PS-Simulink Converter6/LConn1 -- Current Sensor5/RConn1
  Resistor2/LConn1 -- Inductor5/LConn1
  Inductor8/RConn1 -- Resistor1/LConn1
  Inductor8/LConn1 -- Current Sensor8/RConn2
  Current Sensor6/RConn2 -- Inductor9/RConn1
  Subsystem16/RConn1 -- Inductor6/LConn1
  Subsystem16/LConn4 -- PS-Simulink Converter/LConn1
  Subsystem13/LConn4 -- PS-Simulink Converter11/LConn1
  PS-Simulink Converter12/LConn1 -- Subsystem37/LConn4
  PS-Simulink Converter13/LConn1 -- Subsystem7/LConn4
  PS-Simulink Converter14/LConn1 -- Subsystem47/LConn4
  Subsystem54/LConn4 -- PS-Simulink Converter15/LConn1
  Subsystem38/LConn4 -- PS-Simulink Converter16/LConn1
  Subsystem48/LConn4 -- PS-Simulink Converter17/LConn1
  PS-Simulink Converter18/LConn1 -- Subsystem21/LConn4
  Subsystem45/LConn4 -- PS-Simulink Converter19/LConn1
  Subsystem19/LConn4 -- PS-Simulink Converter20/LConn1
  Subsystem43/LConn4 -- PS-Simulink Converter21/LConn1
  Subsystem23/LConn4 -- PS-Simulink Converter22/LConn1
  Subsystem49/LConn4 -- PS-Simulink Converter23/LConn1
  Subsystem20/LConn4 -- PS-Simulink Converter24/LConn1
  Subsystem44/LConn4 -- PS-Simulink Converter25/LConn1
  Subsystem27/LConn4 -- PS-Simulink Converter26/LConn1
  Subsystem52/LConn4 -- PS-Simulink Converter27/LConn1
  Subsystem18/LConn4 -- PS-Simulink Converter28/LConn1
  Subsystem42/LConn4 -- PS-Simulink Converter29/LConn1
  Subsystem3/LConn4 -- PS-Simulink Converter30/LConn1
  Subsystem30/LConn4 -- PS-Simulink Converter31/LConn1
  Subsystem9/LConn4 -- PS-Simulink Converter32/LConn1
  Subsystem33/LConn4 -- PS-Simulink Converter33/LConn1
  Subsystem8/LConn4 -- PS-Simulink Converter34/LConn1
  Subsystem34/LConn4 -- PS-Simulink Converter35/LConn1
  Subsystem53/LConn4 -- PS-Simulink Converter36/LConn1
  Subsystem24/LConn4 -- PS-Simulink Converter38/LConn1
  Subsystem11/LConn4 -- PS-Simulink Converter37/LConn1
  Subsystem39/LConn4 -- PS-Simulink Converter39/LConn1
  Subsystem6/LConn4 -- PS-Simulink Converter40/LConn1
  Subsystem31/LConn4 -- PS-Simulink Converter41/LConn1
  Subsystem51/LConn4 -- PS-Simulink Converter42/LConn1
  Subsystem12/LConn4 -- PS-Simulink Converter43/LConn1
  Subsystem25/LConn4 -- PS-Simulink Converter44/LConn1
  Subsystem40/LConn4 -- PS-Simulink Converter45/LConn1
  Subsystem10/LConn4 -- PS-Simulink Converter46/LConn1
  PS-Simulink Converter47/LConn1 -- Subsystem22/LConn4
  Subsystem36/LConn4 -- PS-Simulink Converter48/LConn1
  Subsystem17/LConn4 -- PS-Simulink Converter49/LConn1
  Subsystem26/LConn4 -- PS-Simulink Converter50/LConn1
  Subsystem41/LConn4 -- PS-Simulink Converter51/LConn1
  Subsystem2/LConn4 -- PS-Simulink Converter52/LConn1
  Subsystem28/LConn4 -- PS-Simulink Converter53/LConn1
  Subsystem46/LConn4 -- PS-Simulink Converter54/LConn1
  Subsystem1/LConn4 -- PS-Simulink Converter55/LConn1
  Subsystem14/LConn4 -- PS-Simulink Converter56/LConn1
  PS-Simulink Converter57/LConn1 -- Subsystem35/LConn4
